simulink model "cmult_core"  (R2013a)
settings: Solver=ode45  StartTime=0.0  StopTime=10.0  RelTol=1e-3
libraries: xbsIndex_r4 x2035, casper_library_misc x116, casper_library_multipliers x36
(part 2 of 23)

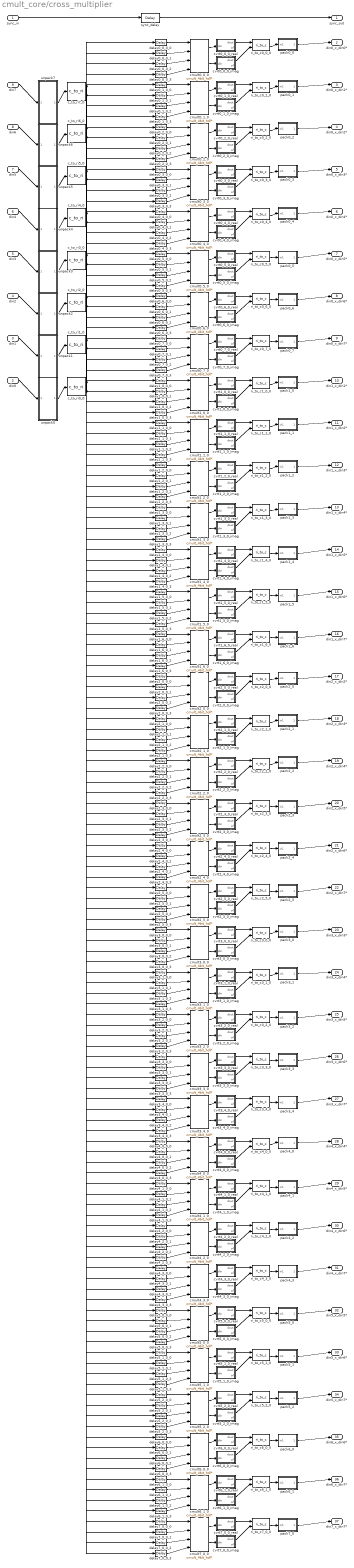
== system cmult_core/cross_multiplier ==
  sync_in : Inport
  din0 : Inport  Port=2
  din1 : Inport  Port=3
  din2 : Inport  Port=4
  din3 : Inport  Port=5
  din4 : Inport  Port=6
  din5 : Inport  Port=7
  din6 : Inport  Port=8
  din7 : Inport  Port=9
  c_to_ri0_0 : casper_library_misc/c_to_ri  n_bits=bit_width_in  bin_pt=binary_point_in
      settings: AttributesFormatString=8_7 r/i
  c_to_ri1_0 : casper_library_misc/c_to_ri  n_bits=bit_width_in  bin_pt=binary_point_in
      settings: AttributesFormatString=8_7 r/i
  c_to_ri2_0 : casper_library_misc/c_to_ri  n_bits=bit_width_in  bin_pt=binary_point_in
      settings: AttributesFormatString=8_7 r/i
  c_to_ri3_0 : casper_library_misc/c_to_ri  n_bits=bit_width_in  bin_pt=binary_point_in
      settings: AttributesFormatString=8_7 r/i
  c_to_ri4_0 : casper_library_misc/c_to_ri  n_bits=bit_width_in  bin_pt=binary_point_in
      settings: AttributesFormatString=8_7 r/i
  c_to_ri5_0 : casper_library_misc/c_to_ri  n_bits=bit_width_in  bin_pt=binary_point_in
      settings: AttributesFormatString=8_7 r/i
  c_to_ri6_0 : casper_library_misc/c_to_ri  n_bits=bit_width_in  bin_pt=binary_point_in
      settings: AttributesFormatString=8_7 r/i
  c_to_ri7_0 : casper_library_misc/c_to_ri  n_bits=bit_width_in  bin_pt=binary_point_in
      settings: AttributesFormatString=8_7 r/i
  cmult0_0_0 : casper_library_multipliers/cmult_4bit_hdl*  mult_latency=mult_latency  add_latency=add_latency
  cmult0_1_0 : casper_library_multipliers/cmult_4bit_hdl*  mult_latency=mult_latency  add_latency=add_latency
  cmult0_2_0 : casper_library_multipliers/cmult_4bit_hdl*  mult_latency=mult_latency  add_latency=add_latency
  cmult0_3_0 : casper_library_multipliers/cmult_4bit_hdl*  mult_latency=mult_latency  add_latency=add_latency
  cmult0_4_0 : casper_library_multipliers/cmult_4bit_hdl*  mult_latency=mult_latency  add_latency=add_latency
  cmult0_5_0 : casper_library_multipliers/cmult_4bit_hdl*  mult_latency=mult_latency  add_latency=add_latency
  cmult0_6_0 : casper_library_multipliers/cmult_4bit_hdl*  mult_latency=mult_latency  add_latency=add_latency
  cmult0_7_0 : casper_library_multipliers/cmult_4bit_hdl*  mult_latency=mult_latency  add_latency=add_latency
  cmult1_0_0 : casper_library_multipliers/cmult_4bit_hdl*  mult_latency=mult_latency  add_latency=add_latency
  cmult1_1_0 : casper_library_multipliers/cmult_4bit_hdl*  mult_latency=mult_latency  add_latency=add_latency
  cmult1_2_0 : casper_library_multipliers/cmult_4bit_hdl*  mult_latency=mult_latency  add_latency=add_latency
  cmult1_3_0 : casper_library_multipliers/cmult_4bit_hdl*  mult_latency=mult_latency  add_latency=add_latency
  cmult1_4_0 : casper_library_multipliers/cmult_4bit_hdl*  mult_latency=mult_latency  add_latency=add_latency
  cmult1_5_0 : casper_library_multipliers/cmult_4bit_hdl*  mult_latency=mult_latency  add_latency=add_latency
  cmult1_6_0 : casper_library_multipliers/cmult_4bit_hdl*  mult_latency=mult_latency  add_latency=add_latency
  cmult2_0_0 : casper_library_multipliers/cmult_4bit_hdl*  mult_latency=mult_latency  add_latency=add_latency
  cmult2_1_0 : casper_library_multipliers/cmult_4bit_hdl*  mult_latency=mult_latency  add_latency=add_latency
  cmult2_2_0 : casper_library_multipliers/cmult_4bit_hdl*  mult_latency=mult_latency  add_latency=add_latency
  cmult2_3_0 : casper_library_multipliers/cmult_4bit_hdl*  mult_latency=mult_latency  add_latency=add_latency
  cmult2_4_0 : casper_library_multipliers/cmult_4bit_hdl*  mult_latency=mult_latency  add_latency=add_latency
  cmult2_5_0 : casper_library_multipliers/cmult_4bit_hdl*  mult_latency=mult_latency  add_latency=add_latency
  cmult3_0_0 : casper_library_multipliers/cmult_4bit_hdl*  mult_latency=mult_latency  add_latency=add_latency
  cmult3_1_0 : casper_library_multipliers/cmult_4bit_hdl*  mult_latency=mult_latency  add_latency=add_latency
  cmult3_2_0 : casper_library_multipliers/cmult_4bit_hdl*  mult_latency=mult_latency  add_latency=add_latency
  cmult3_3_0 : casper_library_multipliers/cmult_4bit_hdl*  mult_latency=mult_latency  add_latency=add_latency
  cmult3_4_0 : casper_library_multipliers/cmult_4bit_hdl*  mult_latency=mult_latency  add_latency=add_latency
  cmult4_0_0 : casper_library_multipliers/cmult_4bit_hdl*  mult_latency=mult_latency  add_latency=add_latency
  cmult4_1_0 : casper_library_multipliers/cmult_4bit_hdl*  mult_latency=mult_latency  add_latency=add_latency
  cmult4_2_0 : casper_library_multipliers/cmult_4bit_hdl*  mult_latency=mult_latency  add_latency=add_latency
  cmult4_3_0 : casper_library_multipliers/cmult_4bit_hdl*  mult_latency=mult_latency  add_latency=add_latency
  cmult5_0_0 : casper_library_multipliers/cmult_4bit_hdl*  mult_latency=mult_latency  add_latency=add_latency
  cmult5_1_0 : casper_library_multipliers/cmult_4bit_hdl*  mult_latency=mult_latency  add_latency=add_latency
  cmult5_2_0 : casper_library_multipliers/cmult_4bit_hdl*  mult_latency=mult_latency  add_latency=add_latency
  cmult6_0_0 : casper_library_multipliers/cmult_4bit_hdl*  mult_latency=mult_latency  add_latency=add_latency
  cmult6_1_0 : casper_library_multipliers/cmult_4bit_hdl*  mult_latency=mult_latency  add_latency=add_latency
  cmult7_0_0 : casper_library_multipliers/cmult_4bit_hdl*  mult_latency=mult_latency  add_latency=add_latency
  cvrt0_0_0_imag : Subsystem  AncestorBlock=casper_library_misc/convert_of  mask(convert_of){bit_width_i=17, binary_point_i=14, bit_width_o=17, binary_point_o=14, latency=0, adder_imp=Fabric, overflow=Wrap, quantization=Truncate}
      mask prompts: bit_width_i "Bit Width In"; binary_point_i "Binary Point In"; bit_width_o "Bit Width Out"; binary_point_o "Binary Point Out"; adder_imp "Adder Implementation"; overflow "Overflow Behaviour"; quantization "Quantization Behaviour"
      mask help:
      | Converts from one 2's complement bit-width
      | and/or binary point position to another.
      | Includes underflow/overflow indicator.
      mask init:
      | convert_of_init(gcb, ...
      |     'bit_width_i', bit_width_i, ...
      |     'binary_point_i', binary_point_i, ...
      |     'bit_width_o', bit_width_o, ...
      |     'binary_point_o', binary_point_o, ...
      |     'latency', latency, ...
      |     'adder_imp', adder_imp, ...
      |     'overflow', overflow, ...
      |     'quantization', quantization);
      settings: AttributesFormatString=[17,14]->[17,14]
      mask TypeOptions adder_imp: Fabric | DSP48 | Behavioural | Xilinx Cast Block
      mask TypeOptions overflow: Wrap | Saturate | Error
      mask TypeOptions quantization: Truncate | Round  (unbiased: +/- Inf) | Round  (unbiased: even values)
  cvrt0_0_0_real : Subsystem  AncestorBlock=casper_library_misc/convert_of  mask(convert_of){bit_width_i=17, binary_point_i=14, bit_width_o=17, binary_point_o=14, latency=0, adder_imp=Fabric, overflow=Wrap, quantization=Truncate}
      mask prompts: bit_width_i "Bit Width In"; binary_point_i "Binary Point In"; bit_width_o "Bit Width Out"; binary_point_o "Binary Point Out"; adder_imp "Adder Implementation"; overflow "Overflow Behaviour"; quantization "Quantization Behaviour"
      mask help:
      | Converts from one 2's complement bit-width
      | and/or binary point position to another.
      | Includes underflow/overflow indicator.
      mask init: same as cmult_core/cross_multiplier/cvrt0_0_0_imag
      settings: AttributesFormatString=[17,14]->[17,14]
      mask TypeOptions adder_imp: Fabric | DSP48 | Behavioural | Xilinx Cast Block
      mask TypeOptions overflow: Wrap | Saturate | Error
      mask TypeOptions quantization: Truncate | Round  (unbiased: +/- Inf) | Round  (unbiased: even values)
  cvrt0_1_0_imag : Subsystem  AncestorBlock=casper_library_misc/convert_of  mask(convert_of){bit_width_i=17, binary_point_i=14, bit_width_o=17, binary_point_o=14, latency=0, adder_imp=Fabric, overflow=Wrap, quantization=Truncate}
      mask prompts: bit_width_i "Bit Width In"; binary_point_i "Binary Point In"; bit_width_o "Bit Width Out"; binary_point_o "Binary Point Out"; adder_imp "Adder Implementation"; overflow "Overflow Behaviour"; quantization "Quantization Behaviour"
      mask help:
      | Converts from one 2's complement bit-width
      | and/or binary point position to another.
      | Includes underflow/overflow indicator.
      mask init: same as cmult_core/cross_multiplier/cvrt0_0_0_imag
      settings: AttributesFormatString=[17,14]->[17,14]
      mask TypeOptions adder_imp: Fabric | DSP48 | Behavioural | Xilinx Cast Block
      mask TypeOptions overflow: Wrap | Saturate | Error
      mask TypeOptions quantization: Truncate | Round  (unbiased: +/- Inf) | Round  (unbiased: even values)
  cvrt0_1_0_real : Subsystem  AncestorBlock=casper_library_misc/convert_of  mask(convert_of){bit_width_i=17, binary_point_i=14, bit_width_o=17, binary_point_o=14, latency=0, adder_imp=Fabric, overflow=Wrap, quantization=Truncate}
      mask prompts: bit_width_i "Bit Width In"; binary_point_i "Binary Point In"; bit_width_o "Bit Width Out"; binary_point_o "Binary Point Out"; adder_imp "Adder Implementation"; overflow "Overflow Behaviour"; quantization "Quantization Behaviour"
      mask help:
      | Converts from one 2's complement bit-width
      | and/or binary point position to another.
      | Includes underflow/overflow indicator.
      mask init: same as cmult_core/cross_multiplier/cvrt0_0_0_imag
      settings: AttributesFormatString=[17,14]->[17,14]
      mask TypeOptions adder_imp: Fabric | DSP48 | Behavioural | Xilinx Cast Block
      mask TypeOptions overflow: Wrap | Saturate | Error
      mask TypeOptions quantization: Truncate | Round  (unbiased: +/- Inf) | Round  (unbiased: even values)
  cvrt0_2_0_imag : Subsystem  AncestorBlock=casper_library_misc/convert_of  mask(convert_of){bit_width_i=17, binary_point_i=14, bit_width_o=17, binary_point_o=14, latency=0, adder_imp=Fabric, overflow=Wrap, quantization=Truncate}
      mask prompts: bit_width_i "Bit Width In"; binary_point_i "Binary Point In"; bit_width_o "Bit Width Out"; binary_point_o "Binary Point Out"; adder_imp "Adder Implementation"; overflow "Overflow Behaviour"; quantization "Quantization Behaviour"
      mask help:
      | Converts from one 2's complement bit-width
      | and/or binary point position to another.
      | Includes underflow/overflow indicator.
      mask init: same as cmult_core/cross_multiplier/cvrt0_0_0_imag
      settings: AttributesFormatString=[17,14]->[17,14]
      mask TypeOptions adder_imp: Fabric | DSP48 | Behavioural | Xilinx Cast Block
      mask TypeOptions overflow: Wrap | Saturate | Error
      mask TypeOptions quantization: Truncate | Round  (unbiased: +/- Inf) | Round  (unbiased: even values)
  cvrt0_2_0_real : Subsystem  AncestorBlock=casper_library_misc/convert_of  mask(convert_of){bit_width_i=17, binary_point_i=14, bit_width_o=17, binary_point_o=14, latency=0, adder_imp=Fabric, overflow=Wrap, quantization=Truncate}
      mask prompts: bit_width_i "Bit Width In"; binary_point_i "Binary Point In"; bit_width_o "Bit Width Out"; binary_point_o "Binary Point Out"; adder_imp "Adder Implementation"; overflow "Overflow Behaviour"; quantization "Quantization Behaviour"
      mask help:
      | Converts from one 2's complement bit-width
      | and/or binary point position to another.
      | Includes underflow/overflow indicator.
      mask init: same as cmult_core/cross_multiplier/cvrt0_0_0_imag
      settings: AttributesFormatString=[17,14]->[17,14]
      mask TypeOptions adder_imp: Fabric | DSP48 | Behavioural | Xilinx Cast Block
      mask TypeOptions overflow: Wrap | Saturate | Error
      mask TypeOptions quantization: Truncate | Round  (unbiased: +/- Inf) | Round  (unbiased: even values)
  cvrt0_3_0_imag : Subsystem  AncestorBlock=casper_library_misc/convert_of  mask(convert_of){bit_width_i=17, binary_point_i=14, bit_width_o=17, binary_point_o=14, latency=0, adder_imp=Fabric, overflow=Wrap, quantization=Truncate}
      mask prompts: bit_width_i "Bit Width In"; binary_point_i "Binary Point In"; bit_width_o "Bit Width Out"; binary_point_o "Binary Point Out"; adder_imp "Adder Implementation"; overflow "Overflow Behaviour"; quantization "Quantization Behaviour"
      mask help:
      | Converts from one 2's complement bit-width
      | and/or binary point position to another.
      | Includes underflow/overflow indicator.
      mask init: same as cmult_core/cross_multiplier/cvrt0_0_0_imag
      settings: AttributesFormatString=[17,14]->[17,14]
      mask TypeOptions adder_imp: Fabric | DSP48 | Behavioural | Xilinx Cast Block
      mask TypeOptions overflow: Wrap | Saturate | Error
      mask TypeOptions quantization: Truncate | Round  (unbiased: +/- Inf) | Round  (unbiased: even values)
  cvrt0_3_0_real : Subsystem  AncestorBlock=casper_library_misc/convert_of  mask(convert_of){bit_width_i=17, binary_point_i=14, bit_width_o=17, binary_point_o=14, latency=0, adder_imp=Fabric, overflow=Wrap, quantization=Truncate}
      mask prompts: bit_width_i "Bit Width In"; binary_point_i "Binary Point In"; bit_width_o "Bit Width Out"; binary_point_o "Binary Point Out"; adder_imp "Adder Implementation"; overflow "Overflow Behaviour"; quantization "Quantization Behaviour"
      mask help:
      | Converts from one 2's complement bit-width
      | and/or binary point position to another.
      | Includes underflow/overflow indicator.
      mask init: same as cmult_core/cross_multiplier/cvrt0_0_0_imag
      settings: AttributesFormatString=[17,14]->[17,14]
      mask TypeOptions adder_imp: Fabric | DSP48 | Behavioural | Xilinx Cast Block
      mask TypeOptions overflow: Wrap | Saturate | Error
      mask TypeOptions quantization: Truncate | Round  (unbiased: +/- Inf) | Round  (unbiased: even values)
  cvrt0_4_0_imag : Subsystem  AncestorBlock=casper_library_misc/convert_of  mask(convert_of){bit_width_i=17, binary_point_i=14, bit_width_o=17, binary_point_o=14, latency=0, adder_imp=Fabric, overflow=Wrap, quantization=Truncate}
      mask prompts: bit_width_i "Bit Width In"; binary_point_i "Binary Point In"; bit_width_o "Bit Width Out"; binary_point_o "Binary Point Out"; adder_imp "Adder Implementation"; overflow "Overflow Behaviour"; quantization "Quantization Behaviour"
      mask help:
      | Converts from one 2's complement bit-width
      | and/or binary point position to another.
      | Includes underflow/overflow indicator.
      mask init: same as cmult_core/cross_multiplier/cvrt0_0_0_imag
      settings: AttributesFormatString=[17,14]->[17,14]
      mask TypeOptions adder_imp: Fabric | DSP48 | Behavioural | Xilinx Cast Block
      mask TypeOptions overflow: Wrap | Saturate | Error
      mask TypeOptions quantization: Truncate | Round  (unbiased: +/- Inf) | Round  (unbiased: even values)
  cvrt0_4_0_real : Subsystem  AncestorBlock=casper_library_misc/convert_of  mask(convert_of){bit_width_i=17, binary_point_i=14, bit_width_o=17, binary_point_o=14, latency=0, adder_imp=Fabric, overflow=Wrap, quantization=Truncate}
      mask prompts: bit_width_i "Bit Width In"; binary_point_i "Binary Point In"; bit_width_o "Bit Width Out"; binary_point_o "Binary Point Out"; adder_imp "Adder Implementation"; overflow "Overflow Behaviour"; quantization "Quantization Behaviour"
      mask help:
      | Converts from one 2's complement bit-width
      | and/or binary point position to another.
      | Includes underflow/overflow indicator.
      mask init: same as cmult_core/cross_multiplier/cvrt0_0_0_imag
      settings: AttributesFormatString=[17,14]->[17,14]
      mask TypeOptions adder_imp: Fabric | DSP48 | Behavioural | Xilinx Cast Block
      mask TypeOptions overflow: Wrap | Saturate | Error
      mask TypeOptions quantization: Truncate | Round  (unbiased: +/- Inf) | Round  (unbiased: even values)
  cvrt0_5_0_imag : Subsystem  AncestorBlock=casper_library_misc/convert_of  mask(convert_of){bit_width_i=17, binary_point_i=14, bit_width_o=17, binary_point_o=14, latency=0, adder_imp=Fabric, overflow=Wrap, quantization=Truncate}
      mask prompts: bit_width_i "Bit Width In"; binary_point_i "Binary Point In"; bit_width_o "Bit Width Out"; binary_point_o "Binary Point Out"; adder_imp "Adder Implementation"; overflow "Overflow Behaviour"; quantization "Quantization Behaviour"
      mask help:
      | Converts from one 2's complement bit-width
      | and/or binary point position to another.
      | Includes underflow/overflow indicator.
      mask init: same as cmult_core/cross_multiplier/cvrt0_0_0_imag
      settings: AttributesFormatString=[17,14]->[17,14]
      mask TypeOptions adder_imp: Fabric | DSP48 | Behavioural | Xilinx Cast Block
      mask TypeOptions overflow: Wrap | Saturate | Error
      mask TypeOptions quantization: Truncate | Round  (unbiased: +/- Inf) | Round  (unbiased: even values)
  cvrt0_5_0_real : Subsystem  AncestorBlock=casper_library_misc/convert_of  mask(convert_of){bit_width_i=17, binary_point_i=14, bit_width_o=17, binary_point_o=14, latency=0, adder_imp=Fabric, overflow=Wrap, quantization=Truncate}
      mask prompts: bit_width_i "Bit Width In"; binary_point_i "Binary Point In"; bit_width_o "Bit Width Out"; binary_point_o "Binary Point Out"; adder_imp "Adder Implementation"; overflow "Overflow Behaviour"; quantization "Quantization Behaviour"
      mask help:
      | Converts from one 2's complement bit-width
      | and/or binary point position to another.
      | Includes underflow/overflow indicator.
      mask init: same as cmult_core/cross_multiplier/cvrt0_0_0_imag
      settings: AttributesFormatString=[17,14]->[17,14]
      mask TypeOptions adder_imp: Fabric | DSP48 | Behavioural | Xilinx Cast Block
      mask TypeOptions overflow: Wrap | Saturate | Error
      mask TypeOptions quantization: Truncate | Round  (unbiased: +/- Inf) | Round  (unbiased: even values)
  cvrt0_6_0_imag : Subsystem  AncestorBlock=casper_library_misc/convert_of  mask(convert_of){bit_width_i=17, binary_point_i=14, bit_width_o=17, binary_point_o=14, latency=0, adder_imp=Fabric, overflow=Wrap, quantization=Truncate}
      mask prompts: bit_width_i "Bit Width In"; binary_point_i "Binary Point In"; bit_width_o "Bit Width Out"; binary_point_o "Binary Point Out"; adder_imp "Adder Implementation"; overflow "Overflow Behaviour"; quantization "Quantization Behaviour"
      mask help:
      | Converts from one 2's complement bit-width
      | and/or binary point position to another.
      | Includes underflow/overflow indicator.
      mask init: same as cmult_core/cross_multiplier/cvrt0_0_0_imag
      settings: AttributesFormatString=[17,14]->[17,14]
      mask TypeOptions adder_imp: Fabric | DSP48 | Behavioural | Xilinx Cast Block
      mask TypeOptions overflow: Wrap | Saturate | Error
      mask TypeOptions quantization: Truncate | Round  (unbiased: +/- Inf) | Round  (unbiased: even values)
  cvrt0_6_0_real : Subsystem  AncestorBlock=casper_library_misc/convert_of  mask(convert_of){bit_width_i=17, binary_point_i=14, bit_width_o=17, binary_point_o=14, latency=0, adder_imp=Fabric, overflow=Wrap, quantization=Truncate}
      mask prompts: bit_width_i "Bit Width In"; binary_point_i "Binary Point In"; bit_width_o "Bit Width Out"; binary_point_o "Binary Point Out"; adder_imp "Adder Implementation"; overflow "Overflow Behaviour"; quantization "Quantization Behaviour"
      mask help:
      | Converts from one 2's complement bit-width
      | and/or binary point position to another.
      | Includes underflow/overflow indicator.
      mask init: same as cmult_core/cross_multiplier/cvrt0_0_0_imag
      settings: AttributesFormatString=[17,14]->[17,14]
      mask TypeOptions adder_imp: Fabric | DSP48 | Behavioural | Xilinx Cast Block
      mask TypeOptions overflow: Wrap | Saturate | Error
      mask TypeOptions quantization: Truncate | Round  (unbiased: +/- Inf) | Round  (unbiased: even values)
  cvrt0_7_0_imag : Subsystem  AncestorBlock=casper_library_misc/convert_of  mask(convert_of){bit_width_i=17, binary_point_i=14, bit_width_o=17, binary_point_o=14, latency=0, adder_imp=Fabric, overflow=Wrap, quantization=Truncate}
      mask prompts: bit_width_i "Bit Width In"; binary_point_i "Binary Point In"; bit_width_o "Bit Width Out"; binary_point_o "Binary Point Out"; adder_imp "Adder Implementation"; overflow "Overflow Behaviour"; quantization "Quantization Behaviour"
      mask help:
      | Converts from one 2's complement bit-width
      | and/or binary point position to another.
      | Includes underflow/overflow indicator.
      mask init: same as cmult_core/cross_multiplier/cvrt0_0_0_imag
      settings: AttributesFormatString=[17,14]->[17,14]
      mask TypeOptions adder_imp: Fabric | DSP48 | Behavioural | Xilinx Cast Block
      mask TypeOptions overflow: Wrap | Saturate | Error
      mask TypeOptions quantization: Truncate | Round  (unbiased: +/- Inf) | Round  (unbiased: even values)
  cvrt0_7_0_real : Subsystem  AncestorBlock=casper_library_misc/convert_of  mask(convert_of){bit_width_i=17, binary_point_i=14, bit_width_o=17, binary_point_o=14, latency=0, adder_imp=Fabric, overflow=Wrap, quantization=Truncate}
      mask prompts: bit_width_i "Bit Width In"; binary_point_i "Binary Point In"; bit_width_o "Bit Width Out"; binary_point_o "Binary Point Out"; adder_imp "Adder Implementation"; overflow "Overflow Behaviour"; quantization "Quantization Behaviour"
      mask help:
      | Converts from one 2's complement bit-width
      | and/or binary point position to another.
      | Includes underflow/overflow indicator.
      mask init: same as cmult_core/cross_multiplier/cvrt0_0_0_imag
      settings: AttributesFormatString=[17,14]->[17,14]
      mask TypeOptions adder_imp: Fabric | DSP48 | Behavioural | Xilinx Cast Block
      mask TypeOptions overflow: Wrap | Saturate | Error
      mask TypeOptions quantization: Truncate | Round  (unbiased: +/- Inf) | Round  (unbiased: even values)
  cvrt1_0_0_imag : Subsystem  AncestorBlock=casper_library_misc/convert_of  mask(convert_of){bit_width_i=17, binary_point_i=14, bit_width_o=17, binary_point_o=14, latency=0, adder_imp=Fabric, overflow=Wrap, quantization=Truncate}
      mask prompts: bit_width_i "Bit Width In"; binary_point_i "Binary Point In"; bit_width_o "Bit Width Out"; binary_point_o "Binary Point Out"; adder_imp "Adder Implementation"; overflow "Overflow Behaviour"; quantization "Quantization Behaviour"
      mask help:
      | Converts from one 2's complement bit-width
      | and/or binary point position to another.
      | Includes underflow/overflow indicator.
      mask init: same as cmult_core/cross_multiplier/cvrt0_0_0_imag
      settings: AttributesFormatString=[17,14]->[17,14]
      mask TypeOptions adder_imp: Fabric | DSP48 | Behavioural | Xilinx Cast Block
      mask TypeOptions overflow: Wrap | Saturate | Error
      mask TypeOptions quantization: Truncate | Round  (unbiased: +/- Inf) | Round  (unbiased: even values)
  cvrt1_0_0_real : Subsystem  AncestorBlock=casper_library_misc/convert_of  mask(convert_of){bit_width_i=17, binary_point_i=14, bit_width_o=17, binary_point_o=14, latency=0, adder_imp=Fabric, overflow=Wrap, quantization=Truncate}
      mask prompts: bit_width_i "Bit Width In"; binary_point_i "Binary Point In"; bit_width_o "Bit Width Out"; binary_point_o "Binary Point Out"; adder_imp "Adder Implementation"; overflow "Overflow Behaviour"; quantization "Quantization Behaviour"
      mask help:
      | Converts from one 2's complement bit-width
      | and/or binary point position to another.
      | Includes underflow/overflow indicator.
      mask init: same as cmult_core/cross_multiplier/cvrt0_0_0_imag
      settings: AttributesFormatString=[17,14]->[17,14]
      mask TypeOptions adder_imp: Fabric | DSP48 | Behavioural | Xilinx Cast Block
      mask TypeOptions overflow: Wrap | Saturate | Error
      mask TypeOptions quantization: Truncate | Round  (unbiased: +/- Inf) | Round  (unbiased: even values)
  cvrt1_1_0_imag : Subsystem  AncestorBlock=casper_library_misc/convert_of  mask(convert_of){bit_width_i=17, binary_point_i=14, bit_width_o=17, binary_point_o=14, latency=0, adder_imp=Fabric, overflow=Wrap, quantization=Truncate}
      mask prompts: bit_width_i "Bit Width In"; binary_point_i "Binary Point In"; bit_width_o "Bit Width Out"; binary_point_o "Binary Point Out"; adder_imp "Adder Implementation"; overflow "Overflow Behaviour"; quantization "Quantization Behaviour"
      mask help:
      | Converts from one 2's complement bit-width
      | and/or binary point position to another.
      | Includes underflow/overflow indicator.
      mask init: same as cmult_core/cross_multiplier/cvrt0_0_0_imag
      settings: AttributesFormatString=[17,14]->[17,14]
      mask TypeOptions adder_imp: Fabric | DSP48 | Behavioural | Xilinx Cast Block
      mask TypeOptions overflow: Wrap | Saturate | Error
      mask TypeOptions quantization: Truncate | Round  (unbiased: +/- Inf) | Round  (unbiased: even values)
  cvrt1_1_0_real : Subsystem  AncestorBlock=casper_library_misc/convert_of  mask(convert_of){bit_width_i=17, binary_point_i=14, bit_width_o=17, binary_point_o=14, latency=0, adder_imp=Fabric, overflow=Wrap, quantization=Truncate}
      mask prompts: bit_width_i "Bit Width In"; binary_point_i "Binary Point In"; bit_width_o "Bit Width Out"; binary_point_o "Binary Point Out"; adder_imp "Adder Implementation"; overflow "Overflow Behaviour"; quantization "Quantization Behaviour"
      mask help:
      | Converts from one 2's complement bit-width
      | and/or binary point position to another.
      | Includes underflow/overflow indicator.
      mask init: same as cmult_core/cross_multiplier/cvrt0_0_0_imag
      settings: AttributesFormatString=[17,14]->[17,14]
      mask TypeOptions adder_imp: Fabric | DSP48 | Behavioural | Xilinx Cast Block
      mask TypeOptions overflow: Wrap | Saturate | Error
      mask TypeOptions quantization: Truncate | Round  (unbiased: +/- Inf) | Round  (unbiased: even values)
  cvrt1_2_0_imag : Subsystem  AncestorBlock=casper_library_misc/convert_of  mask(convert_of){bit_width_i=17, binary_point_i=14, bit_width_o=17, binary_point_o=14, latency=0, adder_imp=Fabric, overflow=Wrap, quantization=Truncate}
      mask prompts: bit_width_i "Bit Width In"; binary_point_i "Binary Point In"; bit_width_o "Bit Width Out"; binary_point_o "Binary Point Out"; adder_imp "Adder Implementation"; overflow "Overflow Behaviour"; quantization "Quantization Behaviour"
      mask help:
      | Converts from one 2's complement bit-width
      | and/or binary point position to another.
      | Includes underflow/overflow indicator.
      mask init: same as cmult_core/cross_multiplier/cvrt0_0_0_imag
      settings: AttributesFormatString=[17,14]->[17,14]
      mask TypeOptions adder_imp: Fabric | DSP48 | Behavioural | Xilinx Cast Block
      mask TypeOptions overflow: Wrap | Saturate | Error
      mask TypeOptions quantization: Truncate | Round  (unbiased: +/- Inf) | Round  (unbiased: even values)
  cvrt1_2_0_real : Subsystem  AncestorBlock=casper_library_misc/convert_of  mask(convert_of){bit_width_i=17, binary_point_i=14, bit_width_o=17, binary_point_o=14, latency=0, adder_imp=Fabric, overflow=Wrap, quantization=Truncate}
      mask prompts: bit_width_i "Bit Width In"; binary_point_i "Binary Point In"; bit_width_o "Bit Width Out"; binary_point_o "Binary Point Out"; adder_imp "Adder Implementation"; overflow "Overflow Behaviour"; quantization "Quantization Behaviour"
      mask help:
      | Converts from one 2's complement bit-width
      | and/or binary point position to another.
      | Includes underflow/overflow indicator.
      mask init: same as cmult_core/cross_multiplier/cvrt0_0_0_imag
      settings: AttributesFormatString=[17,14]->[17,14]
      mask TypeOptions adder_imp: Fabric | DSP48 | Behavioural | Xilinx Cast Block
      mask TypeOptions overflow: Wrap | Saturate | Error
      mask TypeOptions quantization: Truncate | Round  (unbiased: +/- Inf) | Round  (unbiased: even values)
  cvrt1_3_0_imag : Subsystem  AncestorBlock=casper_library_misc/convert_of  mask(convert_of){bit_width_i=17, binary_point_i=14, bit_width_o=17, binary_point_o=14, latency=0, adder_imp=Fabric, overflow=Wrap, quantization=Truncate}
      mask prompts: bit_width_i "Bit Width In"; binary_point_i "Binary Point In"; bit_width_o "Bit Width Out"; binary_point_o "Binary Point Out"; adder_imp "Adder Implementation"; overflow "Overflow Behaviour"; quantization "Quantization Behaviour"
      mask help:
      | Converts from one 2's complement bit-width
      | and/or binary point position to another.
      | Includes underflow/overflow indicator.
      mask init: same as cmult_core/cross_multiplier/cvrt0_0_0_imag
      settings: AttributesFormatString=[17,14]->[17,14]
      mask TypeOptions adder_imp: Fabric | DSP48 | Behavioural | Xilinx Cast Block
      mask TypeOptions overflow: Wrap | Saturate | Error
      mask TypeOptions quantization: Truncate | Round  (unbiased: +/- Inf) | Round  (unbiased: even values)
  cvrt1_3_0_real : Subsystem  AncestorBlock=casper_library_misc/convert_of  mask(convert_of){bit_width_i=17, binary_point_i=14, bit_width_o=17, binary_point_o=14, latency=0, adder_imp=Fabric, overflow=Wrap, quantization=Truncate}
      mask prompts: bit_width_i "Bit Width In"; binary_point_i "Binary Point In"; bit_width_o "Bit Width Out"; binary_point_o "Binary Point Out"; adder_imp "Adder Implementation"; overflow "Overflow Behaviour"; quantization "Quantization Behaviour"
      mask help:
      | Converts from one 2's complement bit-width
      | and/or binary point position to another.
      | Includes underflow/overflow indicator.
      mask init: same as cmult_core/cross_multiplier/cvrt0_0_0_imag
      settings: AttributesFormatString=[17,14]->[17,14]
      mask TypeOptions adder_imp: Fabric | DSP48 | Behavioural | Xilinx Cast Block
      mask TypeOptions overflow: Wrap | Saturate | Error
      mask TypeOptions quantization: Truncate | Round  (unbiased: +/- Inf) | Round  (unbiased: even values)
  cvrt1_4_0_imag : Subsystem  AncestorBlock=casper_library_misc/convert_of  mask(convert_of){bit_width_i=17, binary_point_i=14, bit_width_o=17, binary_point_o=14, latency=0, adder_imp=Fabric, overflow=Wrap, quantization=Truncate}
      mask prompts: bit_width_i "Bit Width In"; binary_point_i "Binary Point In"; bit_width_o "Bit Width Out"; binary_point_o "Binary Point Out"; adder_imp "Adder Implementation"; overflow "Overflow Behaviour"; quantization "Quantization Behaviour"
      mask help:
      | Converts from one 2's complement bit-width
      | and/or binary point position to another.
      | Includes underflow/overflow indicator.
      mask init: same as cmult_core/cross_multiplier/cvrt0_0_0_imag
      settings: AttributesFormatString=[17,14]->[17,14]
      mask TypeOptions adder_imp: Fabric | DSP48 | Behavioural | Xilinx Cast Block
      mask TypeOptions overflow: Wrap | Saturate | Error
      mask TypeOptions quantization: Truncate | Round  (unbiased: +/- Inf) | Round  (unbiased: even values)
  cvrt1_4_0_real : Subsystem  AncestorBlock=casper_library_misc/convert_of  mask(convert_of){bit_width_i=17, binary_point_i=14, bit_width_o=17, binary_point_o=14, latency=0, adder_imp=Fabric, overflow=Wrap, quantization=Truncate}
      mask prompts: bit_width_i "Bit Width In"; binary_point_i "Binary Point In"; bit_width_o "Bit Width Out"; binary_point_o "Binary Point Out"; adder_imp "Adder Implementation"; overflow "Overflow Behaviour"; quantization "Quantization Behaviour"
      mask help:
      | Converts from one 2's complement bit-width
      | and/or binary point position to another.
      | Includes underflow/overflow indicator.
      mask init: same as cmult_core/cross_multiplier/cvrt0_0_0_imag
      settings: AttributesFormatString=[17,14]->[17,14]
      mask TypeOptions adder_imp: Fabric | DSP48 | Behavioural | Xilinx Cast Block
      mask TypeOptions overflow: Wrap | Saturate | Error
      mask TypeOptions quantization: Truncate | Round  (unbiased: +/- Inf) | Round  (unbiased: even values)
  cvrt1_5_0_imag : Subsystem  AncestorBlock=casper_library_misc/convert_of  mask(convert_of){bit_width_i=17, binary_point_i=14, bit_width_o=17, binary_point_o=14, latency=0, adder_imp=Fabric, overflow=Wrap, quantization=Truncate}
      mask prompts: bit_width_i "Bit Width In"; binary_point_i "Binary Point In"; bit_width_o "Bit Width Out"; binary_point_o "Binary Point Out"; adder_imp "Adder Implementation"; overflow "Overflow Behaviour"; quantization "Quantization Behaviour"
      mask help:
      | Converts from one 2's complement bit-width
      | and/or binary point position to another.
      | Includes underflow/overflow indicator.
      mask init: same as cmult_core/cross_multiplier/cvrt0_0_0_imag
      settings: AttributesFormatString=[17,14]->[17,14]
      mask TypeOptions adder_imp: Fabric | DSP48 | Behavioural | Xilinx Cast Block
      mask TypeOptions overflow: Wrap | Saturate | Error
      mask TypeOptions quantization: Truncate | Round  (unbiased: +/- Inf) | Round  (unbiased: even values)
  cvrt1_5_0_real : Subsystem  AncestorBlock=casper_library_misc/convert_of  mask(convert_of){bit_width_i=17, binary_point_i=14, bit_width_o=17, binary_point_o=14, latency=0, adder_imp=Fabric, overflow=Wrap, quantization=Truncate}
      mask prompts: bit_width_i "Bit Width In"; binary_point_i "Binary Point In"; bit_width_o "Bit Width Out"; binary_point_o "Binary Point Out"; adder_imp "Adder Implementation"; overflow "Overflow Behaviour"; quantization "Quantization Behaviour"
      mask help:
      | Converts from one 2's complement bit-width
      | and/or binary point position to another.
      | Includes underflow/overflow indicator.
      mask init: same as cmult_core/cross_multiplier/cvrt0_0_0_imag
      settings: AttributesFormatString=[17,14]->[17,14]
      mask TypeOptions adder_imp: Fabric | DSP48 | Behavioural | Xilinx Cast Block
      mask TypeOptions overflow: Wrap | Saturate | Error
      mask TypeOptions quantization: Truncate | Round  (unbiased: +/- Inf) | Round  (unbiased: even values)
  cvrt1_6_0_imag : Subsystem  AncestorBlock=casper_library_misc/convert_of  mask(convert_of){bit_width_i=17, binary_point_i=14, bit_width_o=17, binary_point_o=14, latency=0, adder_imp=Fabric, overflow=Wrap, quantization=Truncate}
      mask prompts: bit_width_i "Bit Width In"; binary_point_i "Binary Point In"; bit_width_o "Bit Width Out"; binary_point_o "Binary Point Out"; adder_imp "Adder Implementation"; overflow "Overflow Behaviour"; quantization "Quantization Behaviour"
      mask help:
      | Converts from one 2's complement bit-width
      | and/or binary point position to another.
      | Includes underflow/overflow indicator.
      mask init: same as cmult_core/cross_multiplier/cvrt0_0_0_imag
      settings: AttributesFormatString=[17,14]->[17,14]
      mask TypeOptions adder_imp: Fabric | DSP48 | Behavioural | Xilinx Cast Block
      mask TypeOptions overflow: Wrap | Saturate | Error
      mask TypeOptions quantization: Truncate | Round  (unbiased: +/- Inf) | Round  (unbiased: even values)
  cvrt1_6_0_real : Subsystem  AncestorBlock=casper_library_misc/convert_of  mask(convert_of){bit_width_i=17, binary_point_i=14, bit_width_o=17, binary_point_o=14, latency=0, adder_imp=Fabric, overflow=Wrap, quantization=Truncate}
      mask prompts: bit_width_i "Bit Width In"; binary_point_i "Binary Point In"; bit_width_o "Bit Width Out"; binary_point_o "Binary Point Out"; adder_imp "Adder Implementation"; overflow "Overflow Behaviour"; quantization "Quantization Behaviour"
      mask help:
      | Converts from one 2's complement bit-width
      | and/or binary point position to another.
      | Includes underflow/overflow indicator.
      mask init: same as cmult_core/cross_multiplier/cvrt0_0_0_imag
      settings: AttributesFormatString=[17,14]->[17,14]
      mask TypeOptions adder_imp: Fabric | DSP48 | Behavioural | Xilinx Cast Block
      mask TypeOptions overflow: Wrap | Saturate | Error
      mask TypeOptions quantization: Truncate | Round  (unbiased: +/- Inf) | Round  (unbiased: even values)
  cvrt2_0_0_imag : Subsystem  AncestorBlock=casper_library_misc/convert_of  mask(convert_of){bit_width_i=17, binary_point_i=14, bit_width_o=17, binary_point_o=14, latency=0, adder_imp=Fabric, overflow=Wrap, quantization=Truncate}
      mask prompts: bit_width_i "Bit Width In"; binary_point_i "Binary Point In"; bit_width_o "Bit Width Out"; binary_point_o "Binary Point Out"; adder_imp "Adder Implementation"; overflow "Overflow Behaviour"; quantization "Quantization Behaviour"
      mask help:
      | Converts from one 2's complement bit-width
      | and/or binary point position to another.
      | Includes underflow/overflow indicator.
      mask init: same as cmult_core/cross_multiplier/cvrt0_0_0_imag
      settings: AttributesFormatString=[17,14]->[17,14]
      mask TypeOptions adder_imp: Fabric | DSP48 | Behavioural | Xilinx Cast Block
      mask TypeOptions overflow: Wrap | Saturate | Error
      mask TypeOptions quantization: Truncate | Round  (unbiased: +/- Inf) | Round  (unbiased: even values)
  cvrt2_0_0_real : Subsystem  AncestorBlock=casper_library_misc/convert_of  mask(convert_of){bit_width_i=17, binary_point_i=14, bit_width_o=17, binary_point_o=14, latency=0, adder_imp=Fabric, overflow=Wrap, quantization=Truncate}
      mask prompts: bit_width_i "Bit Width In"; binary_point_i "Binary Point In"; bit_width_o "Bit Width Out"; binary_point_o "Binary Point Out"; adder_imp "Adder Implementation"; overflow "Overflow Behaviour"; quantization "Quantization Behaviour"
      mask help:
      | Converts from one 2's complement bit-width
      | and/or binary point position to another.
      | Includes underflow/overflow indicator.
      mask init: same as cmult_core/cross_multiplier/cvrt0_0_0_imag
      settings: AttributesFormatString=[17,14]->[17,14]
      mask TypeOptions adder_imp: Fabric | DSP48 | Behavioural | Xilinx Cast Block
      mask TypeOptions overflow: Wrap | Saturate | Error
      mask TypeOptions quantization: Truncate | Round  (unbiased: +/- Inf) | Round  (unbiased: even values)
  cvrt2_1_0_imag : Subsystem  AncestorBlock=casper_library_misc/convert_of  mask(convert_of){bit_width_i=17, binary_point_i=14, bit_width_o=17, binary_point_o=14, latency=0, adder_imp=Fabric, overflow=Wrap, quantization=Truncate}
      mask prompts: bit_width_i "Bit Width In"; binary_point_i "Binary Point In"; bit_width_o "Bit Width Out"; binary_point_o "Binary Point Out"; adder_imp "Adder Implementation"; overflow "Overflow Behaviour"; quantization "Quantization Behaviour"
      mask help:
      | Converts from one 2's complement bit-width
      | and/or binary point position to another.
      | Includes underflow/overflow indicator.
      mask init: same as cmult_core/cross_multiplier/cvrt0_0_0_imag
      settings: AttributesFormatString=[17,14]->[17,14]
      mask TypeOptions adder_imp: Fabric | DSP48 | Behavioural | Xilinx Cast Block
      mask TypeOptions overflow: Wrap | Saturate | Error
      mask TypeOptions quantization: Truncate | Round  (unbiased: +/- Inf) | Round  (unbiased: even values)
  cvrt2_1_0_real : Subsystem  AncestorBlock=casper_library_misc/convert_of  mask(convert_of){bit_width_i=17, binary_point_i=14, bit_width_o=17, binary_point_o=14, latency=0, adder_imp=Fabric, overflow=Wrap, quantization=Truncate}
      mask prompts: bit_width_i "Bit Width In"; binary_point_i "Binary Point In"; bit_width_o "Bit Width Out"; binary_point_o "Binary Point Out"; adder_imp "Adder Implementation"; overflow "Overflow Behaviour"; quantization "Quantization Behaviour"
      mask help:
      | Converts from one 2's complement bit-width
      | and/or binary point position to another.
      | Includes underflow/overflow indicator.
      mask init: same as cmult_core/cross_multiplier/cvrt0_0_0_imag
      settings: AttributesFormatString=[17,14]->[17,14]
      mask TypeOptions adder_imp: Fabric | DSP48 | Behavioural | Xilinx Cast Block
      mask TypeOptions overflow: Wrap | Saturate | Error
      mask TypeOptions quantization: Truncate | Round  (unbiased: +/- Inf) | Round  (unbiased: even values)
  cvrt2_2_0_imag : Subsystem  AncestorBlock=casper_library_misc/convert_of  mask(convert_of){bit_width_i=17, binary_point_i=14, bit_width_o=17, binary_point_o=14, latency=0, adder_imp=Fabric, overflow=Wrap, quantization=Truncate}
      mask prompts: bit_width_i "Bit Width In"; binary_point_i "Binary Point In"; bit_width_o "Bit Width Out"; binary_point_o "Binary Point Out"; adder_imp "Adder Implementation"; overflow "Overflow Behaviour"; quantization "Quantization Behaviour"
      mask help:
      | Converts from one 2's complement bit-width
      | and/or binary point position to another.
      | Includes underflow/overflow indicator.
      mask init: same as cmult_core/cross_multiplier/cvrt0_0_0_imag
      settings: AttributesFormatString=[17,14]->[17,14]
      mask TypeOptions adder_imp: Fabric | DSP48 | Behavioural | Xilinx Cast Block
      mask TypeOptions overflow: Wrap | Saturate | Error
      mask TypeOptions quantization: Truncate | Round  (unbiased: +/- Inf) | Round  (unbiased: even values)
  cvrt2_2_0_real : Subsystem  AncestorBlock=casper_library_misc/convert_of  mask(convert_of){bit_width_i=17, binary_point_i=14, bit_width_o=17, binary_point_o=14, latency=0, adder_imp=Fabric, overflow=Wrap, quantization=Truncate}
      mask prompts: bit_width_i "Bit Width In"; binary_point_i "Binary Point In"; bit_width_o "Bit Width Out"; binary_point_o "Binary Point Out"; adder_imp "Adder Implementation"; overflow "Overflow Behaviour"; quantization "Quantization Behaviour"
      mask help:
      | Converts from one 2's complement bit-width
      | and/or binary point position to another.
      | Includes underflow/overflow indicator.
      mask init: same as cmult_core/cross_multiplier/cvrt0_0_0_imag
      settings: AttributesFormatString=[17,14]->[17,14]
      mask TypeOptions adder_imp: Fabric | DSP48 | Behavioural | Xilinx Cast Block
      mask TypeOptions overflow: Wrap | Saturate | Error
      mask TypeOptions quantization: Truncate | Round  (unbiased: +/- Inf) | Round  (unbiased: even values)
  cvrt2_3_0_imag : Subsystem  AncestorBlock=casper_library_misc/convert_of  mask(convert_of){bit_width_i=17, binary_point_i=14, bit_width_o=17, binary_point_o=14, latency=0, adder_imp=Fabric, overflow=Wrap, quantization=Truncate}
      mask prompts: bit_width_i "Bit Width In"; binary_point_i "Binary Point In"; bit_width_o "Bit Width Out"; binary_point_o "Binary Point Out"; adder_imp "Adder Implementation"; overflow "Overflow Behaviour"; quantization "Quantization Behaviour"
      mask help:
      | Converts from one 2's complement bit-width
      | and/or binary point position to another.
      | Includes underflow/overflow indicator.
      mask init: same as cmult_core/cross_multiplier/cvrt0_0_0_imag
      settings: AttributesFormatString=[17,14]->[17,14]
      mask TypeOptions adder_imp: Fabric | DSP48 | Behavioural | Xilinx Cast Block
      mask TypeOptions overflow: Wrap | Saturate | Error
      mask TypeOptions quantization: Truncate | Round  (unbiased: +/- Inf) | Round  (unbiased: even values)
  cvrt2_3_0_real : Subsystem  AncestorBlock=casper_library_misc/convert_of  mask(convert_of){bit_width_i=17, binary_point_i=14, bit_width_o=17, binary_point_o=14, latency=0, adder_imp=Fabric, overflow=Wrap, quantization=Truncate}
      mask prompts: bit_width_i "Bit Width In"; binary_point_i "Binary Point In"; bit_width_o "Bit Width Out"; binary_point_o "Binary Point Out"; adder_imp "Adder Implementation"; overflow "Overflow Behaviour"; quantization "Quantization Behaviour"
      mask help:
      | Converts from one 2's complement bit-width
      | and/or binary point position to another.
      | Includes underflow/overflow indicator.
      mask init: same as cmult_core/cross_multiplier/cvrt0_0_0_imag
      settings: AttributesFormatString=[17,14]->[17,14]
      mask TypeOptions adder_imp: Fabric | DSP48 | Behavioural | Xilinx Cast Block
      mask TypeOptions overflow: Wrap | Saturate | Error
      mask TypeOptions quantization: Truncate | Round  (unbiased: +/- Inf) | Round  (unbiased: even values)
  cvrt2_4_0_imag : Subsystem  AncestorBlock=casper_library_misc/convert_of  mask(convert_of){bit_width_i=17, binary_point_i=14, bit_width_o=17, binary_point_o=14, latency=0, adder_imp=Fabric, overflow=Wrap, quantization=Truncate}
      mask prompts: bit_width_i "Bit Width In"; binary_point_i "Binary Point In"; bit_width_o "Bit Width Out"; binary_point_o "Binary Point Out"; adder_imp "Adder Implementation"; overflow "Overflow Behaviour"; quantization "Quantization Behaviour"
      mask help:
      | Converts from one 2's complement bit-width
      | and/or binary point position to another.
      | Includes underflow/overflow indicator.
      mask init: same as cmult_core/cross_multiplier/cvrt0_0_0_imag
      settings: AttributesFormatString=[17,14]->[17,14]
      mask TypeOptions adder_imp: Fabric | DSP48 | Behavioural | Xilinx Cast Block
      mask TypeOptions overflow: Wrap | Saturate | Error
      mask TypeOptions quantization: Truncate | Round  (unbiased: +/- Inf) | Round  (unbiased: even values)
  cvrt2_4_0_real : Subsystem  AncestorBlock=casper_library_misc/convert_of  mask(convert_of){bit_width_i=17, binary_point_i=14, bit_width_o=17, binary_point_o=14, latency=0, adder_imp=Fabric, overflow=Wrap, quantization=Truncate}
      mask prompts: bit_width_i "Bit Width In"; binary_point_i "Binary Point In"; bit_width_o "Bit Width Out"; binary_point_o "Binary Point Out"; adder_imp "Adder Implementation"; overflow "Overflow Behaviour"; quantization "Quantization Behaviour"
      mask help:
      | Converts from one 2's complement bit-width
      | and/or binary point position to another.
      | Includes underflow/overflow indicator.
      mask init: same as cmult_core/cross_multiplier/cvrt0_0_0_imag
      settings: AttributesFormatString=[17,14]->[17,14]
      mask TypeOptions adder_imp: Fabric | DSP48 | Behavioural | Xilinx Cast Block
      mask TypeOptions overflow: Wrap | Saturate | Error
      mask TypeOptions quantization: Truncate | Round  (unbiased: +/- Inf) | Round  (unbiased: even values)
  cvrt2_5_0_imag : Subsystem  AncestorBlock=casper_library_misc/convert_of  mask(convert_of){bit_width_i=17, binary_point_i=14, bit_width_o=17, binary_point_o=14, latency=0, adder_imp=Fabric, overflow=Wrap, quantization=Truncate}
      mask prompts: bit_width_i "Bit Width In"; binary_point_i "Binary Point In"; bit_width_o "Bit Width Out"; binary_point_o "Binary Point Out"; adder_imp "Adder Implementation"; overflow "Overflow Behaviour"; quantization "Quantization Behaviour"
      mask help:
      | Converts from one 2's complement bit-width
      | and/or binary point position to another.
      | Includes underflow/overflow indicator.
      mask init: same as cmult_core/cross_multiplier/cvrt0_0_0_imag
      settings: AttributesFormatString=[17,14]->[17,14]
      mask TypeOptions adder_imp: Fabric | DSP48 | Behavioural | Xilinx Cast Block
      mask TypeOptions overflow: Wrap | Saturate | Error
      mask TypeOptions quantization: Truncate | Round  (unbiased: +/- Inf) | Round  (unbiased: even values)
  cvrt2_5_0_real : Subsystem  AncestorBlock=casper_library_misc/convert_of  mask(convert_of){bit_width_i=17, binary_point_i=14, bit_width_o=17, binary_point_o=14, latency=0, adder_imp=Fabric, overflow=Wrap, quantization=Truncate}
      mask prompts: bit_width_i "Bit Width In"; binary_point_i "Binary Point In"; bit_width_o "Bit Width Out"; binary_point_o "Binary Point Out"; adder_imp "Adder Implementation"; overflow "Overflow Behaviour"; quantization "Quantization Behaviour"
      mask help:
      | Converts from one 2's complement bit-width
      | and/or binary point position to another.
      | Includes underflow/overflow indicator.
      mask init: same as cmult_core/cross_multiplier/cvrt0_0_0_imag
      settings: AttributesFormatString=[17,14]->[17,14]
      mask TypeOptions adder_imp: Fabric | DSP48 | Behavioural | Xilinx Cast Block
      mask TypeOptions overflow: Wrap | Saturate | Error
      mask TypeOptions quantization: Truncate | Round  (unbiased: +/- Inf) | Round  (unbiased: even values)
  cvrt3_0_0_imag : Subsystem  AncestorBlock=casper_library_misc/convert_of  mask(convert_of){bit_width_i=17, binary_point_i=14, bit_width_o=17, binary_point_o=14, latency=0, adder_imp=Fabric, overflow=Wrap, quantization=Truncate}
      mask prompts: bit_width_i "Bit Width In"; binary_point_i "Binary Point In"; bit_width_o "Bit Width Out"; binary_point_o "Binary Point Out"; adder_imp "Adder Implementation"; overflow "Overflow Behaviour"; quantization "Quantization Behaviour"
      mask help:
      | Converts from one 2's complement bit-width
      | and/or binary point position to another.
      | Includes underflow/overflow indicator.
      mask init: same as cmult_core/cross_multiplier/cvrt0_0_0_imag
      settings: AttributesFormatString=[17,14]->[17,14]
      mask TypeOptions adder_imp: Fabric | DSP48 | Behavioural | Xilinx Cast Block
      mask TypeOptions overflow: Wrap | Saturate | Error
      mask TypeOptions quantization: Truncate | Round  (unbiased: +/- Inf) | Round  (unbiased: even values)
  cvrt3_0_0_real : Subsystem  AncestorBlock=casper_library_misc/convert_of  mask(convert_of){bit_width_i=17, binary_point_i=14, bit_width_o=17, binary_point_o=14, latency=0, adder_imp=Fabric, overflow=Wrap, quantization=Truncate}
      mask prompts: bit_width_i "Bit Width In"; binary_point_i "Binary Point In"; bit_width_o "Bit Width Out"; binary_point_o "Binary Point Out"; adder_imp "Adder Implementation"; overflow "Overflow Behaviour"; quantization "Quantization Behaviour"
      mask help:
      | Converts from one 2's complement bit-width
      | and/or binary point position to another.
      | Includes underflow/overflow indicator.
      mask init: same as cmult_core/cross_multiplier/cvrt0_0_0_imag
      settings: AttributesFormatString=[17,14]->[17,14]
      mask TypeOptions adder_imp: Fabric | DSP48 | Behavioural | Xilinx Cast Block
      mask TypeOptions overflow: Wrap | Saturate | Error
      mask TypeOptions quantization: Truncate | Round  (unbiased: +/- Inf) | Round  (unbiased: even values)
  cvrt3_1_0_imag : Subsystem  AncestorBlock=casper_library_misc/convert_of  mask(convert_of){bit_width_i=17, binary_point_i=14, bit_width_o=17, binary_point_o=14, latency=0, adder_imp=Fabric, overflow=Wrap, quantization=Truncate}
      mask prompts: bit_width_i "Bit Width In"; binary_point_i "Binary Point In"; bit_width_o "Bit Width Out"; binary_point_o "Binary Point Out"; adder_imp "Adder Implementation"; overflow "Overflow Behaviour"; quantization "Quantization Behaviour"
      mask help:
      | Converts from one 2's complement bit-width
      | and/or binary point position to another.
      | Includes underflow/overflow indicator.
      mask init: same as cmult_core/cross_multiplier/cvrt0_0_0_imag
      settings: AttributesFormatString=[17,14]->[17,14]
      mask TypeOptions adder_imp: Fabric | DSP48 | Behavioural | Xilinx Cast Block
      mask TypeOptions overflow: Wrap | Saturate | Error
      mask TypeOptions quantization: Truncate | Round  (unbiased: +/- Inf) | Round  (unbiased: even values)
  cvrt3_1_0_real : Subsystem  AncestorBlock=casper_library_misc/convert_of  mask(convert_of){bit_width_i=17, binary_point_i=14, bit_width_o=17, binary_point_o=14, latency=0, adder_imp=Fabric, overflow=Wrap, quantization=Truncate}
      mask prompts: bit_width_i "Bit Width In"; binary_point_i "Binary Point In"; bit_width_o "Bit Width Out"; binary_point_o "Binary Point Out"; adder_imp "Adder Implementation"; overflow "Overflow Behaviour"; quantization "Quantization Behaviour"
      mask help:
      | Converts from one 2's complement bit-width
      | and/or binary point position to another.
      | Includes underflow/overflow indicator.
      mask init: same as cmult_core/cross_multiplier/cvrt0_0_0_imag
      settings: AttributesFormatString=[17,14]->[17,14]
      mask TypeOptions adder_imp: Fabric | DSP48 | Behavioural | Xilinx Cast Block
      mask TypeOptions overflow: Wrap | Saturate | Error
      mask TypeOptions quantization: Truncate | Round  (unbiased: +/- Inf) | Round  (unbiased: even values)
  cvrt3_2_0_imag : Subsystem  AncestorBlock=casper_library_misc/convert_of  mask(convert_of){bit_width_i=17, binary_point_i=14, bit_width_o=17, binary_point_o=14, latency=0, adder_imp=Fabric, overflow=Wrap, quantization=Truncate}
      mask prompts: bit_width_i "Bit Width In"; binary_point_i "Binary Point In"; bit_width_o "Bit Width Out"; binary_point_o "Binary Point Out"; adder_imp "Adder Implementation"; overflow "Overflow Behaviour"; quantization "Quantization Behaviour"
      mask help:
      | Converts from one 2's complement bit-width
      | and/or binary point position to another.
      | Includes underflow/overflow indicator.
      mask init: same as cmult_core/cross_multiplier/cvrt0_0_0_imag
      settings: AttributesFormatString=[17,14]->[17,14]
      mask TypeOptions adder_imp: Fabric | DSP48 | Behavioural | Xilinx Cast Block
      mask TypeOptions overflow: Wrap | Saturate | Error
      mask TypeOptions quantization: Truncate | Round  (unbiased: +/- Inf) | Round  (unbiased: even values)
  cvrt3_2_0_real : Subsystem  AncestorBlock=casper_library_misc/convert_of  mask(convert_of){bit_width_i=17, binary_point_i=14, bit_width_o=17, binary_point_o=14, latency=0, adder_imp=Fabric, overflow=Wrap, quantization=Truncate}
      mask prompts: bit_width_i "Bit Width In"; binary_point_i "Binary Point In"; bit_width_o "Bit Width Out"; binary_point_o "Binary Point Out"; adder_imp "Adder Implementation"; overflow "Overflow Behaviour"; quantization "Quantization Behaviour"
      mask help:
      | Converts from one 2's complement bit-width
      | and/or binary point position to another.
      | Includes underflow/overflow indicator.
      mask init: same as cmult_core/cross_multiplier/cvrt0_0_0_imag
      settings: AttributesFormatString=[17,14]->[17,14]
      mask TypeOptions adder_imp: Fabric | DSP48 | Behavioural | Xilinx Cast Block
      mask TypeOptions overflow: Wrap | Saturate | Error
      mask TypeOptions quantization: Truncate | Round  (unbiased: +/- Inf) | Round  (unbiased: even values)
  cvrt3_3_0_imag : Subsystem  AncestorBlock=casper_library_misc/convert_of  mask(convert_of){bit_width_i=17, binary_point_i=14, bit_width_o=17, binary_point_o=14, latency=0, adder_imp=Fabric, overflow=Wrap, quantization=Truncate}
      mask prompts: bit_width_i "Bit Width In"; binary_point_i "Binary Point In"; bit_width_o "Bit Width Out"; binary_point_o "Binary Point Out"; adder_imp "Adder Implementation"; overflow "Overflow Behaviour"; quantization "Quantization Behaviour"
      mask help:
      | Converts from one 2's complement bit-width
      | and/or binary point position to another.
      | Includes underflow/overflow indicator.
      mask init: same as cmult_core/cross_multiplier/cvrt0_0_0_imag
      settings: AttributesFormatString=[17,14]->[17,14]
      mask TypeOptions adder_imp: Fabric | DSP48 | Behavioural | Xilinx Cast Block
      mask TypeOptions overflow: Wrap | Saturate | Error
      mask TypeOptions quantization: Truncate | Round  (unbiased: +/- Inf) | Round  (unbiased: even values)
  cvrt3_3_0_real : Subsystem  AncestorBlock=casper_library_misc/convert_of  mask(convert_of){bit_width_i=17, binary_point_i=14, bit_width_o=17, binary_point_o=14, latency=0, adder_imp=Fabric, overflow=Wrap, quantization=Truncate}
      mask prompts: bit_width_i "Bit Width In"; binary_point_i "Binary Point In"; bit_width_o "Bit Width Out"; binary_point_o "Binary Point Out"; adder_imp "Adder Implementation"; overflow "Overflow Behaviour"; quantization "Quantization Behaviour"
      mask help:
      | Converts from one 2's complement bit-width
      | and/or binary point position to another.
      | Includes underflow/overflow indicator.
      mask init: same as cmult_core/cross_multiplier/cvrt0_0_0_imag
      settings: AttributesFormatString=[17,14]->[17,14]
      mask TypeOptions adder_imp: Fabric | DSP48 | Behavioural | Xilinx Cast Block
      mask TypeOptions overflow: Wrap | Saturate | Error
      mask TypeOptions quantization: Truncate | Round  (unbiased: +/- Inf) | Round  (unbiased: even values)
  cvrt3_4_0_imag : Subsystem  AncestorBlock=casper_library_misc/convert_of  mask(convert_of){bit_width_i=17, binary_point_i=14, bit_width_o=17, binary_point_o=14, latency=0, adder_imp=Fabric, overflow=Wrap, quantization=Truncate}
      mask prompts: bit_width_i "Bit Width In"; binary_point_i "Binary Point In"; bit_width_o "Bit Width Out"; binary_point_o "Binary Point Out"; adder_imp "Adder Implementation"; overflow "Overflow Behaviour"; quantization "Quantization Behaviour"
      mask help:
      | Converts from one 2's complement bit-width
      | and/or binary point position to another.
      | Includes underflow/overflow indicator.
      mask init: same as cmult_core/cross_multiplier/cvrt0_0_0_imag
      settings: AttributesFormatString=[17,14]->[17,14]
      mask TypeOptions adder_imp: Fabric | DSP48 | Behavioural | Xilinx Cast Block
      mask TypeOptions overflow: Wrap | Saturate | Error
      mask TypeOptions quantization: Truncate | Round  (unbiased: +/- Inf) | Round  (unbiased: even values)
  cvrt3_4_0_real : Subsystem  AncestorBlock=casper_library_misc/convert_of  mask(convert_of){bit_width_i=17, binary_point_i=14, bit_width_o=17, binary_point_o=14, latency=0, adder_imp=Fabric, overflow=Wrap, quantization=Truncate}
      mask prompts: bit_width_i "Bit Width In"; binary_point_i "Binary Point In"; bit_width_o "Bit Width Out"; binary_point_o "Binary Point Out"; adder_imp "Adder Implementation"; overflow "Overflow Behaviour"; quantization "Quantization Behaviour"
      mask help:
      | Converts from one 2's complement bit-width
      | and/or binary point position to another.
      | Includes underflow/overflow indicator.
      mask init: same as cmult_core/cross_multiplier/cvrt0_0_0_imag
      settings: AttributesFormatString=[17,14]->[17,14]
      mask TypeOptions adder_imp: Fabric | DSP48 | Behavioural | Xilinx Cast Block
      mask TypeOptions overflow: Wrap | Saturate | Error
      mask TypeOptions quantization: Truncate | Round  (unbiased: +/- Inf) | Round  (unbiased: even values)
  cvrt4_0_0_imag : Subsystem  AncestorBlock=casper_library_misc/convert_of  mask(convert_of){bit_width_i=17, binary_point_i=14, bit_width_o=17, binary_point_o=14, latency=0, adder_imp=Fabric, overflow=Wrap, quantization=Truncate}
      mask prompts: bit_width_i "Bit Width In"; binary_point_i "Binary Point In"; bit_width_o "Bit Width Out"; binary_point_o "Binary Point Out"; adder_imp "Adder Implementation"; overflow "Overflow Behaviour"; quantization "Quantization Behaviour"
      mask help:
      | Converts from one 2's complement bit-width
      | and/or binary point position to another.
      | Includes underflow/overflow indicator.
      mask init: same as cmult_core/cross_multiplier/cvrt0_0_0_imag
      settings: AttributesFormatString=[17,14]->[17,14]
      mask TypeOptions adder_imp: Fabric | DSP48 | Behavioural | Xilinx Cast Block
      mask TypeOptions overflow: Wrap | Saturate | Error
      mask TypeOptions quantization: Truncate | Round  (unbiased: +/- Inf) | Round  (unbiased: even values)
  cvrt4_0_0_real : Subsystem  AncestorBlock=casper_library_misc/convert_of  mask(convert_of){bit_width_i=17, binary_point_i=14, bit_width_o=17, binary_point_o=14, latency=0, adder_imp=Fabric, overflow=Wrap, quantization=Truncate}
      mask prompts: bit_width_i "Bit Width In"; binary_point_i "Binary Point In"; bit_width_o "Bit Width Out"; binary_point_o "Binary Point Out"; adder_imp "Adder Implementation"; overflow "Overflow Behaviour"; quantization "Quantization Behaviour"
      mask help:
      | Converts from one 2's complement bit-width
      | and/or binary point position to another.
      | Includes underflow/overflow indicator.
      mask init: same as cmult_core/cross_multiplier/cvrt0_0_0_imag
      settings: AttributesFormatString=[17,14]->[17,14]
      mask TypeOptions adder_imp: Fabric | DSP48 | Behavioural | Xilinx Cast Block
      mask TypeOptions overflow: Wrap | Saturate | Error
      mask TypeOptions quantization: Truncate | Round  (unbiased: +/- Inf) | Round  (unbiased: even values)
  cvrt4_1_0_imag : Subsystem  AncestorBlock=casper_library_misc/convert_of  mask(convert_of){bit_width_i=17, binary_point_i=14, bit_width_o=17, binary_point_o=14, latency=0, adder_imp=Fabric, overflow=Wrap, quantization=Truncate}
      mask prompts: bit_width_i "Bit Width In"; binary_point_i "Binary Point In"; bit_width_o "Bit Width Out"; binary_point_o "Binary Point Out"; adder_imp "Adder Implementation"; overflow "Overflow Behaviour"; quantization "Quantization Behaviour"
      mask help:
      | Converts from one 2's complement bit-width
      | and/or binary point position to another.
      | Includes underflow/overflow indicator.
      mask init: same as cmult_core/cross_multiplier/cvrt0_0_0_imag
      settings: AttributesFormatString=[17,14]->[17,14]
      mask TypeOptions adder_imp: Fabric | DSP48 | Behavioural | Xilinx Cast Block
      mask TypeOptions overflow: Wrap | Saturate | Error
      mask TypeOptions quantization: Truncate | Round  (unbiased: +/- Inf) | Round  (unbiased: even values)
  cvrt4_1_0_real : Subsystem  AncestorBlock=casper_library_misc/convert_of  mask(convert_of){bit_width_i=17, binary_point_i=14, bit_width_o=17, binary_point_o=14, latency=0, adder_imp=Fabric, overflow=Wrap, quantization=Truncate}
      mask prompts: bit_width_i "Bit Width In"; binary_point_i "Binary Point In"; bit_width_o "Bit Width Out"; binary_point_o "Binary Point Out"; adder_imp "Adder Implementation"; overflow "Overflow Behaviour"; quantization "Quantization Behaviour"
      mask help:
      | Converts from one 2's complement bit-width
      | and/or binary point position to another.
      | Includes underflow/overflow indicator.
      mask init: same as cmult_core/cross_multiplier/cvrt0_0_0_imag
      settings: AttributesFormatString=[17,14]->[17,14]
      mask TypeOptions adder_imp: Fabric | DSP48 | Behavioural | Xilinx Cast Block
      mask TypeOptions overflow: Wrap | Saturate | Error
      mask TypeOptions quantization: Truncate | Round  (unbiased: +/- Inf) | Round  (unbiased: even values)
  cvrt4_2_0_imag : Subsystem  AncestorBlock=casper_library_misc/convert_of  mask(convert_of){bit_width_i=17, binary_point_i=14, bit_width_o=17, binary_point_o=14, latency=0, adder_imp=Fabric, overflow=Wrap, quantization=Truncate}
      mask prompts: bit_width_i "Bit Width In"; binary_point_i "Binary Point In"; bit_width_o "Bit Width Out"; binary_point_o "Binary Point Out"; adder_imp "Adder Implementation"; overflow "Overflow Behaviour"; quantization "Quantization Behaviour"
      mask help:
      | Converts from one 2's complement bit-width
      | and/or binary point position to another.
      | Includes underflow/overflow indicator.
      mask init: same as cmult_core/cross_multiplier/cvrt0_0_0_imag
      settings: AttributesFormatString=[17,14]->[17,14]
      mask TypeOptions adder_imp: Fabric | DSP48 | Behavioural | Xilinx Cast Block
      mask TypeOptions overflow: Wrap | Saturate | Error
      mask TypeOptions quantization: Truncate | Round  (unbiased: +/- Inf) | Round  (unbiased: even values)
  cvrt4_2_0_real : Subsystem  AncestorBlock=casper_library_misc/convert_of  mask(convert_of){bit_width_i=17, binary_point_i=14, bit_width_o=17, binary_point_o=14, latency=0, adder_imp=Fabric, overflow=Wrap, quantization=Truncate}
      mask prompts: bit_width_i "Bit Width In"; binary_point_i "Binary Point In"; bit_width_o "Bit Width Out"; binary_point_o "Binary Point Out"; adder_imp "Adder Implementation"; overflow "Overflow Behaviour"; quantization "Quantization Behaviour"
      mask help:
      | Converts from one 2's complement bit-width
      | and/or binary point position to another.
      | Includes underflow/overflow indicator.
      mask init: same as cmult_core/cross_multiplier/cvrt0_0_0_imag
      settings: AttributesFormatString=[17,14]->[17,14]
      mask TypeOptions adder_imp: Fabric | DSP48 | Behavioural | Xilinx Cast Block
      mask TypeOptions overflow: Wrap | Saturate | Error
      mask TypeOptions quantization: Truncate | Round  (unbiased: +/- Inf) | Round  (unbiased: even values)
  cvrt4_3_0_imag : Subsystem  AncestorBlock=casper_library_misc/convert_of  mask(convert_of){bit_width_i=17, binary_point_i=14, bit_width_o=17, binary_point_o=14, latency=0, adder_imp=Fabric, overflow=Wrap, quantization=Truncate}
      mask prompts: bit_width_i "Bit Width In"; binary_point_i "Binary Point In"; bit_width_o "Bit Width Out"; binary_point_o "Binary Point Out"; adder_imp "Adder Implementation"; overflow "Overflow Behaviour"; quantization "Quantization Behaviour"
      mask help:
      | Converts from one 2's complement bit-width
      | and/or binary point position to another.
      | Includes underflow/overflow indicator.
      mask init: same as cmult_core/cross_multiplier/cvrt0_0_0_imag
      settings: AttributesFormatString=[17,14]->[17,14]
      mask TypeOptions adder_imp: Fabric | DSP48 | Behavioural | Xilinx Cast Block
      mask TypeOptions overflow: Wrap | Saturate | Error
      mask TypeOptions quantization: Truncate | Round  (unbiased: +/- Inf) | Round  (unbiased: even values)
  cvrt4_3_0_real : Subsystem  AncestorBlock=casper_library_misc/convert_of  mask(convert_of){bit_width_i=17, binary_point_i=14, bit_width_o=17, binary_point_o=14, latency=0, adder_imp=Fabric, overflow=Wrap, quantization=Truncate}
      mask prompts: bit_width_i "Bit Width In"; binary_point_i "Binary Point In"; bit_width_o "Bit Width Out"; binary_point_o "Binary Point Out"; adder_imp "Adder Implementation"; overflow "Overflow Behaviour"; quantization "Quantization Behaviour"
      mask help:
      | Converts from one 2's complement bit-width
      | and/or binary point position to another.
      | Includes underflow/overflow indicator.
      mask init: same as cmult_core/cross_multiplier/cvrt0_0_0_imag
      settings: AttributesFormatString=[17,14]->[17,14]
      mask TypeOptions adder_imp: Fabric | DSP48 | Behavioural | Xilinx Cast Block
      mask TypeOptions overflow: Wrap | Saturate | Error
      mask TypeOptions quantization: Truncate | Round  (unbiased: +/- Inf) | Round  (unbiased: even values)
  cvrt5_0_0_imag : Subsystem  AncestorBlock=casper_library_misc/convert_of  mask(convert_of){bit_width_i=17, binary_point_i=14, bit_width_o=17, binary_point_o=14, latency=0, adder_imp=Fabric, overflow=Wrap, quantization=Truncate}
      mask prompts: bit_width_i "Bit Width In"; binary_point_i "Binary Point In"; bit_width_o "Bit Width Out"; binary_point_o "Binary Point Out"; adder_imp "Adder Implementation"; overflow "Overflow Behaviour"; quantization "Quantization Behaviour"
      mask help:
      | Converts from one 2's complement bit-width
      | and/or binary point position to another.
      | Includes underflow/overflow indicator.
      mask init: same as cmult_core/cross_multiplier/cvrt0_0_0_imag
      settings: AttributesFormatString=[17,14]->[17,14]
      mask TypeOptions adder_imp: Fabric | DSP48 | Behavioural | Xilinx Cast Block
      mask TypeOptions overflow: Wrap | Saturate | Error
      mask TypeOptions quantization: Truncate | Round  (unbiased: +/- Inf) | Round  (unbiased: even values)
  cvrt5_0_0_real : Subsystem  AncestorBlock=casper_library_misc/convert_of  mask(convert_of){bit_width_i=17, binary_point_i=14, bit_width_o=17, binary_point_o=14, latency=0, adder_imp=Fabric, overflow=Wrap, quantization=Truncate}
      mask prompts: bit_width_i "Bit Width In"; binary_point_i "Binary Point In"; bit_width_o "Bit Width Out"; binary_point_o "Binary Point Out"; adder_imp "Adder Implementation"; overflow "Overflow Behaviour"; quantization "Quantization Behaviour"
      mask help:
      | Converts from one 2's complement bit-width
      | and/or binary point position to another.
      | Includes underflow/overflow indicator.
      mask init: same as cmult_core/cross_multiplier/cvrt0_0_0_imag
      settings: AttributesFormatString=[17,14]->[17,14]
      mask TypeOptions adder_imp: Fabric | DSP48 | Behavioural | Xilinx Cast Block
      mask TypeOptions overflow: Wrap | Saturate | Error
      mask TypeOptions quantization: Truncate | Round  (unbiased: +/- Inf) | Round  (unbiased: even values)
  cvrt5_1_0_imag : Subsystem  AncestorBlock=casper_library_misc/convert_of  mask(convert_of){bit_width_i=17, binary_point_i=14, bit_width_o=17, binary_point_o=14, latency=0, adder_imp=Fabric, overflow=Wrap, quantization=Truncate}
      mask prompts: bit_width_i "Bit Width In"; binary_point_i "Binary Point In"; bit_width_o "Bit Width Out"; binary_point_o "Binary Point Out"; adder_imp "Adder Implementation"; overflow "Overflow Behaviour"; quantization "Quantization Behaviour"
      mask help:
      | Converts from one 2's complement bit-width
      | and/or binary point position to another.
      | Includes underflow/overflow indicator.
      mask init: same as cmult_core/cross_multiplier/cvrt0_0_0_imag
      settings: AttributesFormatString=[17,14]->[17,14]
      mask TypeOptions adder_imp: Fabric | DSP48 | Behavioural | Xilinx Cast Block
      mask TypeOptions overflow: Wrap | Saturate | Error
      mask TypeOptions quantization: Truncate | Round  (unbiased: +/- Inf) | Round  (unbiased: even values)
  cvrt5_1_0_real : Subsystem  AncestorBlock=casper_library_misc/convert_of  mask(convert_of){bit_width_i=17, binary_point_i=14, bit_width_o=17, binary_point_o=14, latency=0, adder_imp=Fabric, overflow=Wrap, quantization=Truncate}
      mask prompts: bit_width_i "Bit Width In"; binary_point_i "Binary Point In"; bit_width_o "Bit Width Out"; binary_point_o "Binary Point Out"; adder_imp "Adder Implementation"; overflow "Overflow Behaviour"; quantization "Quantization Behaviour"
      mask help:
      | Converts from one 2's complement bit-width
      | and/or binary point position to another.
      | Includes underflow/overflow indicator.
      mask init: same as cmult_core/cross_multiplier/cvrt0_0_0_imag
      settings: AttributesFormatString=[17,14]->[17,14]
      mask TypeOptions adder_imp: Fabric | DSP48 | Behavioural | Xilinx Cast Block
      mask TypeOptions overflow: Wrap | Saturate | Error
      mask TypeOptions quantization: Truncate | Round  (unbiased: +/- Inf) | Round  (unbiased: even values)
  cvrt5_2_0_imag : Subsystem  AncestorBlock=casper_library_misc/convert_of  mask(convert_of){bit_width_i=17, binary_point_i=14, bit_width_o=17, binary_point_o=14, latency=0, adder_imp=Fabric, overflow=Wrap, quantization=Truncate}
      mask prompts: bit_width_i "Bit Width In"; binary_point_i "Binary Point In"; bit_width_o "Bit Width Out"; binary_point_o "Binary Point Out"; adder_imp "Adder Implementation"; overflow "Overflow Behaviour"; quantization "Quantization Behaviour"
      mask help:
      | Converts from one 2's complement bit-width
      | and/or binary point position to another.
      | Includes underflow/overflow indicator.
      mask init: same as cmult_core/cross_multiplier/cvrt0_0_0_imag
      settings: AttributesFormatString=[17,14]->[17,14]
      mask TypeOptions adder_imp: Fabric | DSP48 | Behavioural | Xilinx Cast Block
      mask TypeOptions overflow: Wrap | Saturate | Error
      mask TypeOptions quantization: Truncate | Round  (unbiased: +/- Inf) | Round  (unbiased: even values)
  cvrt5_2_0_real : Subsystem  AncestorBlock=casper_library_misc/convert_of  mask(convert_of){bit_width_i=17, binary_point_i=14, bit_width_o=17, binary_point_o=14, latency=0, adder_imp=Fabric, overflow=Wrap, quantization=Truncate}
      mask prompts: bit_width_i "Bit Width In"; binary_point_i "Binary Point In"; bit_width_o "Bit Width Out"; binary_point_o "Binary Point Out"; adder_imp "Adder Implementation"; overflow "Overflow Behaviour"; quantization "Quantization Behaviour"
      mask help:
      | Converts from one 2's complement bit-width
      | and/or binary point position to another.
      | Includes underflow/overflow indicator.
      mask init: same as cmult_core/cross_multiplier/cvrt0_0_0_imag
      settings: AttributesFormatString=[17,14]->[17,14]
      mask TypeOptions adder_imp: Fabric | DSP48 | Behavioural | Xilinx Cast Block
      mask TypeOptions overflow: Wrap | Saturate | Error
      mask TypeOptions quantization: Truncate | Round  (unbiased: +/- Inf) | Round  (unbiased: even values)
  cvrt6_0_0_imag : Subsystem  AncestorBlock=casper_library_misc/convert_of  mask(convert_of){bit_width_i=17, binary_point_i=14, bit_width_o=17, binary_point_o=14, latency=0, adder_imp=Fabric, overflow=Wrap, quantization=Truncate}
      mask prompts: bit_width_i "Bit Width In"; binary_point_i "Binary Point In"; bit_width_o "Bit Width Out"; binary_point_o "Binary Point Out"; adder_imp "Adder Implementation"; overflow "Overflow Behaviour"; quantization "Quantization Behaviour"
      mask help:
      | Converts from one 2's complement bit-width
      | and/or binary point position to another.
      | Includes underflow/overflow indicator.
      mask init: same as cmult_core/cross_multiplier/cvrt0_0_0_imag
      settings: AttributesFormatString=[17,14]->[17,14]
      mask TypeOptions adder_imp: Fabric | DSP48 | Behavioural | Xilinx Cast Block
      mask TypeOptions overflow: Wrap | Saturate | Error
      mask TypeOptions quantization: Truncate | Round  (unbiased: +/- Inf) | Round  (unbiased: even values)
  cvrt6_0_0_real : Subsystem  AncestorBlock=casper_library_misc/convert_of  mask(convert_of){bit_width_i=17, binary_point_i=14, bit_width_o=17, binary_point_o=14, latency=0, adder_imp=Fabric, overflow=Wrap, quantization=Truncate}
      mask prompts: bit_width_i "Bit Width In"; binary_point_i "Binary Point In"; bit_width_o "Bit Width Out"; binary_point_o "Binary Point Out"; adder_imp "Adder Implementation"; overflow "Overflow Behaviour"; quantization "Quantization Behaviour"
      mask help:
      | Converts from one 2's complement bit-width
      | and/or binary point position to another.
      | Includes underflow/overflow indicator.
      mask init: same as cmult_core/cross_multiplier/cvrt0_0_0_imag
      settings: AttributesFormatString=[17,14]->[17,14]
      mask TypeOptions adder_imp: Fabric | DSP48 | Behavioural | Xilinx Cast Block
      mask TypeOptions overflow: Wrap | Saturate | Error
      mask TypeOptions quantization: Truncate | Round  (unbiased: +/- Inf) | Round  (unbiased: even values)
  cvrt6_1_0_imag : Subsystem  AncestorBlock=casper_library_misc/convert_of  mask(convert_of){bit_width_i=17, binary_point_i=14, bit_width_o=17, binary_point_o=14, latency=0, adder_imp=Fabric, overflow=Wrap, quantization=Truncate}
      mask prompts: bit_width_i "Bit Width In"; binary_point_i "Binary Point In"; bit_width_o "Bit Width Out"; binary_point_o "Binary Point Out"; adder_imp "Adder Implementation"; overflow "Overflow Behaviour"; quantization "Quantization Behaviour"
      mask help:
      | Converts from one 2's complement bit-width
      | and/or binary point position to another.
      | Includes underflow/overflow indicator.
      mask init: same as cmult_core/cross_multiplier/cvrt0_0_0_imag
      settings: AttributesFormatString=[17,14]->[17,14]
      mask TypeOptions adder_imp: Fabric | DSP48 | Behavioural | Xilinx Cast Block
      mask TypeOptions overflow: Wrap | Saturate | Error
      mask TypeOptions quantization: Truncate | Round  (unbiased: +/- Inf) | Round  (unbiased: even values)
  cvrt6_1_0_real : Subsystem  AncestorBlock=casper_library_misc/convert_of  mask(convert_of){bit_width_i=17, binary_point_i=14, bit_width_o=17, binary_point_o=14, latency=0, adder_imp=Fabric, overflow=Wrap, quantization=Truncate}
      mask prompts: bit_width_i "Bit Width In"; binary_point_i "Binary Point In"; bit_width_o "Bit Width Out"; binary_point_o "Binary Point Out"; adder_imp "Adder Implementation"; overflow "Overflow Behaviour"; quantization "Quantization Behaviour"
      mask help:
      | Converts from one 2's complement bit-width
      | and/or binary point position to another.
      | Includes underflow/overflow indicator.
      mask init: same as cmult_core/cross_multiplier/cvrt0_0_0_imag
      settings: AttributesFormatString=[17,14]->[17,14]
      mask TypeOptions adder_imp: Fabric | DSP48 | Behavioural | Xilinx Cast Block
      mask TypeOptions overflow: Wrap | Saturate | Error
      mask TypeOptions quantization: Truncate | Round  (unbiased: +/- Inf) | Round  (unbiased: even values)
  cvrt7_0_0_imag : Subsystem  AncestorBlock=casper_library_misc/convert_of  mask(convert_of){bit_width_i=17, binary_point_i=14, bit_width_o=17, binary_point_o=14, latency=0, adder_imp=Fabric, overflow=Wrap, quantization=Truncate}
      mask prompts: bit_width_i "Bit Width In"; binary_point_i "Binary Point In"; bit_width_o "Bit Width Out"; binary_point_o "Binary Point Out"; adder_imp "Adder Implementation"; overflow "Overflow Behaviour"; quantization "Quantization Behaviour"
      mask help:
      | Converts from one 2's complement bit-width
      | and/or binary point position to another.
      | Includes underflow/overflow indicator.
      mask init: same as cmult_core/cross_multiplier/cvrt0_0_0_imag
      settings: AttributesFormatString=[17,14]->[17,14]
      mask TypeOptions adder_imp: Fabric | DSP48 | Behavioural | Xilinx Cast Block
      mask TypeOptions overflow: Wrap | Saturate | Error
      mask TypeOptions quantization: Truncate | Round  (unbiased: +/- Inf) | Round  (unbiased: even values)
  cvrt7_0_0_real : Subsystem  AncestorBlock=casper_library_misc/convert_of  mask(convert_of){bit_width_i=17, binary_point_i=14, bit_width_o=17, binary_point_o=14, latency=0, adder_imp=Fabric, overflow=Wrap, quantization=Truncate}
      mask prompts: bit_width_i "Bit Width In"; binary_point_i "Binary Point In"; bit_width_o "Bit Width Out"; binary_point_o "Binary Point Out"; adder_imp "Adder Implementation"; overflow "Overflow Behaviour"; quantization "Quantization Behaviour"
      mask help:
      | Converts from one 2's complement bit-width
      | and/or binary point position to another.
      | Includes underflow/overflow indicator.
      mask init: same as cmult_core/cross_multiplier/cvrt0_0_0_imag
      settings: AttributesFormatString=[17,14]->[17,14]
      mask TypeOptions adder_imp: Fabric | DSP48 | Behavioural | Xilinx Cast Block
      mask TypeOptions overflow: Wrap | Saturate | Error
      mask TypeOptions quantization: Truncate | Round  (unbiased: +/- Inf) | Round  (unbiased: even values)
  delay0_0_0_{0..3} (4 alike) : xbsIndex_r4/Delay  rst=off  infoeditControl=Selection of Reset will increase slice count due to use of real FFs and instead of SRLs  en=off  latency=1  dbl_ovrd=off  reg_retiming=off  block_type=delay
  delay0_1_0_{0..3} (4 alike) : xbsIndex_r4/Delay  rst=off  infoeditControl=Selection of Reset will increase slice count due to use of real FFs and instead of SRLs  en=off  latency=1  dbl_ovrd=off  reg_retiming=off  block_type=delay
  delay0_2_0_{0..3} (4 alike) : xbsIndex_r4/Delay  rst=off  infoeditControl=Selection of Reset will increase slice count due to use of real FFs and instead of SRLs  en=off  latency=1  dbl_ovrd=off  reg_retiming=off  block_type=delay
  delay0_3_0_{0..3} (4 alike) : xbsIndex_r4/Delay  rst=off  infoeditControl=Selection of Reset will increase slice count due to use of real FFs and instead of SRLs  en=off  latency=1  dbl_ovrd=off  reg_retiming=off  block_type=delay
  delay0_4_0_{0..3} (4 alike) : xbsIndex_r4/Delay  rst=off  infoeditControl=Selection of Reset will increase slice count due to use of real FFs and instead of SRLs  en=off  latency=1  dbl_ovrd=off  reg_retiming=off  block_type=delay
  delay0_5_0_{0..3} (4 alike) : xbsIndex_r4/Delay  rst=off  infoeditControl=Selection of Reset will increase slice count due to use of real FFs and instead of SRLs  en=off  latency=1  dbl_ovrd=off  reg_retiming=off  block_type=delay
  delay0_6_0_{0..3} (4 alike) : xbsIndex_r4/Delay  rst=off  infoeditControl=Selection of Reset will increase slice count due to use of real FFs and instead of SRLs  en=off  latency=1  dbl_ovrd=off  reg_retiming=off  block_type=delay
  delay0_7_0_{0..3} (4 alike) : xbsIndex_r4/Delay  rst=off  infoeditControl=Selection of Reset will increase slice count due to use of real FFs and instead of SRLs  en=off  latency=1  dbl_ovrd=off  reg_retiming=off  block_type=delay
  delay1_0_0_{0..3} (4 alike) : xbsIndex_r4/Delay  rst=off  infoeditControl=Selection of Reset will increase slice count due to use of real FFs and instead of SRLs  en=off  latency=1  dbl_ovrd=off  reg_retiming=off  block_type=delay
  delay1_1_0_{0..3} (4 alike) : xbsIndex_r4/Delay  rst=off  infoeditControl=Selection of Reset will increase slice count due to use of real FFs and instead of SRLs  en=off  latency=1  dbl_ovrd=off  reg_retiming=off  block_type=delay
  delay1_2_0_{0..3} (4 alike) : xbsIndex_r4/Delay  rst=off  infoeditControl=Selection of Reset will increase slice count due to use of real FFs and instead of SRLs  en=off  latency=1  dbl_ovrd=off  reg_retiming=off  block_type=delay
  delay1_3_0_{0..3} (4 alike) : xbsIndex_r4/Delay  rst=off  infoeditControl=Selection of Reset will increase slice count due to use of real FFs and instead of SRLs  en=off  latency=1  dbl_ovrd=off  reg_retiming=off  block_type=delay
  delay1_4_0_{0..3} (4 alike) : xbsIndex_r4/Delay  rst=off  infoeditControl=Selection of Reset will increase slice count due to use of real FFs and instead of SRLs  en=off  latency=1  dbl_ovrd=off  reg_retiming=off  block_type=delay
  delay1_5_0_{0..3} (4 alike) : xbsIndex_r4/Delay  rst=off  infoeditControl=Selection of Reset will increase slice count due to use of real FFs and instead of SRLs  en=off  latency=1  dbl_ovrd=off  reg_retiming=off  block_type=delay
  delay1_6_0_{0..3} (4 alike) : xbsIndex_r4/Delay  rst=off  infoeditControl=Selection of Reset will increase slice count due to use of real FFs and instead of SRLs  en=off  latency=1  dbl_ovrd=off  reg_retiming=off  block_type=delay
  delay2_0_0_{0..3} (4 alike) : xbsIndex_r4/Delay  rst=off  infoeditControl=Selection of Reset will increase slice count due to use of real FFs and instead of SRLs  en=off  latency=1  dbl_ovrd=off  reg_retiming=off  block_type=delay
  delay2_1_0_{0..3} (4 alike) : xbsIndex_r4/Delay  rst=off  infoeditControl=Selection of Reset will increase slice count due to use of real FFs and instead of SRLs  en=off  latency=1  dbl_ovrd=off  reg_retiming=off  block_type=delay
  delay2_2_0_{0..3} (4 alike) : xbsIndex_r4/Delay  rst=off  infoeditControl=Selection of Reset will increase slice count due to use of real FFs and instead of SRLs  en=off  latency=1  dbl_ovrd=off  reg_retiming=off  block_type=delay
  delay2_3_0_{0..3} (4 alike) : xbsIndex_r4/Delay  rst=off  infoeditControl=Selection of Reset will increase slice count due to use of real FFs and instead of SRLs  en=off  latency=1  dbl_ovrd=off  reg_retiming=off  block_type=delay
  delay2_4_0_{0..3} (4 alike) : xbsIndex_r4/Delay  rst=off  infoeditControl=Selection of Reset will increase slice count due to use of real FFs and instead of SRLs  en=off  latency=1  dbl_ovrd=off  reg_retiming=off  block_type=delay
  delay2_5_0_{0..3} (4 alike) : xbsIndex_r4/Delay  rst=off  infoeditControl=Selection of Reset will increase slice count due to use of real FFs and instead of SRLs  en=off  latency=1  dbl_ovrd=off  reg_retiming=off  block_type=delay
  delay3_0_0_{0..3} (4 alike) : xbsIndex_r4/Delay  rst=off  infoeditControl=Selection of Reset will increase slice count due to use of real FFs and instead of SRLs  en=off  latency=1  dbl_ovrd=off  reg_retiming=off  block_type=delay
  delay3_1_0_{0..3} (4 alike) : xbsIndex_r4/Delay  rst=off  infoeditControl=Selection of Reset will increase slice count due to use of real FFs and instead of SRLs  en=off  latency=1  dbl_ovrd=off  reg_retiming=off  block_type=delay
  delay3_2_0_{0..3} (4 alike) : xbsIndex_r4/Delay  rst=off  infoeditControl=Selection of Reset will increase slice count due to use of real FFs and instead of SRLs  en=off  latency=1  dbl_ovrd=off  reg_retiming=off  block_type=delay
  delay3_3_0_{0..3} (4 alike) : xbsIndex_r4/Delay  rst=off  infoeditControl=Selection of Reset will increase slice count due to use of real FFs and instead of SRLs  en=off  latency=1  dbl_ovrd=off  reg_retiming=off  block_type=delay
  delay3_4_0_{0..3} (4 alike) : xbsIndex_r4/Delay  rst=off  infoeditControl=Selection of Reset will increase slice count due to use of real FFs and instead of SRLs  en=off  latency=1  dbl_ovrd=off  reg_retiming=off  block_type=delay
  delay4_0_0_{0..3} (4 alike) : xbsIndex_r4/Delay  rst=off  infoeditControl=Selection of Reset will increase slice count due to use of real FFs and instead of SRLs  en=off  latency=1  dbl_ovrd=off  reg_retiming=off  block_type=delay
  delay4_1_0_{0..3} (4 alike) : xbsIndex_r4/Delay  rst=off  infoeditControl=Selection of Reset will increase slice count due to use of real FFs and instead of SRLs  en=off  latency=1  dbl_ovrd=off  reg_retiming=off  block_type=delay
  delay4_2_0_{0..3} (4 alike) : xbsIndex_r4/Delay  rst=off  infoeditControl=Selection of Reset will increase slice count due to use of real FFs and instead of SRLs  en=off  latency=1  dbl_ovrd=off  reg_retiming=off  block_type=delay
  delay4_3_0_{0..3} (4 alike) : xbsIndex_r4/Delay  rst=off  infoeditControl=Selection of Reset will increase slice count due to use of real FFs and instead of SRLs  en=off  latency=1  dbl_ovrd=off  reg_retiming=off  block_type=delay
  delay5_0_0_{0..3} (4 alike) : xbsIndex_r4/Delay  rst=off  infoeditControl=Selection of Reset will increase slice count due to use of real FFs and instead of SRLs  en=off  latency=1  dbl_ovrd=off  reg_retiming=off  block_type=delay
  delay5_1_0_{0..3} (4 alike) : xbsIndex_r4/Delay  rst=off  infoeditControl=Selection of Reset will increase slice count due to use of real FFs and instead of SRLs  en=off  latency=1  dbl_ovrd=off  reg_retiming=off  block_type=delay
  delay5_2_0_{0..3} (4 alike) : xbsIndex_r4/Delay  rst=off  infoeditControl=Selection of Reset will increase slice count due to use of real FFs and instead of SRLs  en=off  latency=1  dbl_ovrd=off  reg_retiming=off  block_type=delay
  delay6_0_0_{0..3} (4 alike) : xbsIndex_r4/Delay  rst=off  infoeditControl=Selection of Reset will increase slice count due to use of real FFs and instead of SRLs  en=off  latency=1  dbl_ovrd=off  reg_retiming=off  block_type=delay
  delay6_1_0_{0..3} (4 alike) : xbsIndex_r4/Delay  rst=off  infoeditControl=Selection of Reset will increase slice count due to use of real FFs and instead of SRLs  en=off  latency=1  dbl_ovrd=off  reg_retiming=off  block_type=delay
  delay7_0_0_{0..3} (4 alike) : xbsIndex_r4/Delay  rst=off  infoeditControl=Selection of Reset will increase slice count due to use of real FFs and instead of SRLs  en=off  latency=1  dbl_ovrd=off  reg_retiming=off  block_type=delay
  pack0_0 : Subsystem  AncestorBlock=casper_library_flow_control/bus_create  mask(bus_create){inputNum=aggregation}
      mask prompts: inputNum "Number of inputs:"
      mask init:
      | bus_create_init(gcb,...
      |     'inputNum', inputNum);
  pack0_1 : Subsystem  AncestorBlock=casper_library_flow_control/bus_create  mask(bus_create){inputNum=aggregation}
      mask prompts: inputNum "Number of inputs:"
      mask init:
      | bus_create_init(gcb,...
      |     'inputNum', inputNum);
  pack0_2 : Subsystem  AncestorBlock=casper_library_flow_control/bus_create  mask(bus_create){inputNum=aggregation}
      mask prompts: inputNum "Number of inputs:"
      mask init:
      | bus_create_init(gcb,...
      |     'inputNum', inputNum);
  pack0_3 : Subsystem  AncestorBlock=casper_library_flow_control/bus_create  mask(bus_create){inputNum=aggregation}
      mask prompts: inputNum "Number of inputs:"
      mask init:
      | bus_create_init(gcb,...
      |     'inputNum', inputNum);
  pack0_4 : Subsystem  AncestorBlock=casper_library_flow_control/bus_create  mask(bus_create){inputNum=aggregation}
      mask prompts: inputNum "Number of inputs:"
      mask init:
      | bus_create_init(gcb,...
      |     'inputNum', inputNum);
  pack0_5 : Subsystem  AncestorBlock=casper_library_flow_control/bus_create  mask(bus_create){inputNum=aggregation}
      mask prompts: inputNum "Number of inputs:"
      mask init:
      | bus_create_init(gcb,...
      |     'inputNum', inputNum);
  pack0_6 : Subsystem  AncestorBlock=casper_library_flow_control/bus_create  mask(bus_create){inputNum=aggregation}
      mask prompts: inputNum "Number of inputs:"
      mask init:
      | bus_create_init(gcb,...
      |     'inputNum', inputNum);
  pack0_7 : Subsystem  AncestorBlock=casper_library_flow_control/bus_create  mask(bus_create){inputNum=aggregation}
      mask prompts: inputNum "Number of inputs:"
      mask init:
      | bus_create_init(gcb,...
      |     'inputNum', inputNum);
  pack1_0 : Subsystem  AncestorBlock=casper_library_flow_control/bus_create  mask(bus_create){inputNum=aggregation}
      mask prompts: inputNum "Number of inputs:"
      mask init:
      | bus_create_init(gcb,...
      |     'inputNum', inputNum);
  pack1_1 : Subsystem  AncestorBlock=casper_library_flow_control/bus_create  mask(bus_create){inputNum=aggregation}
      mask prompts: inputNum "Number of inputs:"
      mask init:
      | bus_create_init(gcb,...
      |     'inputNum', inputNum);
  pack1_2 : Subsystem  AncestorBlock=casper_library_flow_control/bus_create  mask(bus_create){inputNum=aggregation}
      mask prompts: inputNum "Number of inputs:"
      mask init:
      | bus_create_init(gcb,...
      |     'inputNum', inputNum);
  pack1_3 : Subsystem  AncestorBlock=casper_library_flow_control/bus_create  mask(bus_create){inputNum=aggregation}
      mask prompts: inputNum "Number of inputs:"
      mask init:
      | bus_create_init(gcb,...
      |     'inputNum', inputNum);
  pack1_4 : Subsystem  AncestorBlock=casper_library_flow_control/bus_create  mask(bus_create){inputNum=aggregation}
      mask prompts: inputNum "Number of inputs:"
      mask init:
      | bus_create_init(gcb,...
      |     'inputNum', inputNum);
  pack1_5 : Subsystem  AncestorBlock=casper_library_flow_control/bus_create  mask(bus_create){inputNum=aggregation}
      mask prompts: inputNum "Number of inputs:"
      mask init:
      | bus_create_init(gcb,...
      |     'inputNum', inputNum);
  pack1_6 : Subsystem  AncestorBlock=casper_library_flow_control/bus_create  mask(bus_create){inputNum=aggregation}
      mask prompts: inputNum "Number of inputs:"
      mask init:
      | bus_create_init(gcb,...
      |     'inputNum', inputNum);
  pack2_0 : Subsystem  AncestorBlock=casper_library_flow_control/bus_create  mask(bus_create){inputNum=aggregation}
      mask prompts: inputNum "Number of inputs:"
      mask init:
      | bus_create_init(gcb,...
      |     'inputNum', inputNum);
  pack2_1 : Subsystem  AncestorBlock=casper_library_flow_control/bus_create  mask(bus_create){inputNum=aggregation}
      mask prompts: inputNum "Number of inputs:"
      mask init:
      | bus_create_init(gcb,...
      |     'inputNum', inputNum);
  pack2_2 : Subsystem  AncestorBlock=casper_library_flow_control/bus_create  mask(bus_create){inputNum=aggregation}
      mask prompts: inputNum "Number of inputs:"
      mask init:
      | bus_create_init(gcb,...
      |     'inputNum', inputNum);
  pack2_3 : Subsystem  AncestorBlock=casper_library_flow_control/bus_create  mask(bus_create){inputNum=aggregation}
      mask prompts: inputNum "Number of inputs:"
      mask init:
      | bus_create_init(gcb,...
      |     'inputNum', inputNum);
  pack2_4 : Subsystem  AncestorBlock=casper_library_flow_control/bus_create  mask(bus_create){inputNum=aggregation}
      mask prompts: inputNum "Number of inputs:"
      mask init:
      | bus_create_init(gcb,...
      |     'inputNum', inputNum);
  pack2_5 : Subsystem  AncestorBlock=casper_library_flow_control/bus_create  mask(bus_create){inputNum=aggregation}
      mask prompts: inputNum "Number of inputs:"
      mask init:
      | bus_create_init(gcb,...
      |     'inputNum', inputNum);
  pack3_0 : Subsystem  AncestorBlock=casper_library_flow_control/bus_create  mask(bus_create){inputNum=aggregation}
      mask prompts: inputNum "Number of inputs:"
      mask init:
      | bus_create_init(gcb,...
      |     'inputNum', inputNum);
  pack3_1 : Subsystem  AncestorBlock=casper_library_flow_control/bus_create  mask(bus_create){inputNum=aggregation}
      mask prompts: inputNum "Number of inputs:"
      mask init:
      | bus_create_init(gcb,...
      |     'inputNum', inputNum);
  pack3_2 : Subsystem  AncestorBlock=casper_library_flow_control/bus_create  mask(bus_create){inputNum=aggregation}
      mask prompts: inputNum "Number of inputs:"
      mask init:
      | bus_create_init(gcb,...
      |     'inputNum', inputNum);
  pack3_3 : Subsystem  AncestorBlock=casper_library_flow_control/bus_create  mask(bus_create){inputNum=aggregation}
      mask prompts: inputNum "Number of inputs:"
      mask init:
      | bus_create_init(gcb,...
      |     'inputNum', inputNum);
  pack3_4 : Subsystem  AncestorBlock=casper_library_flow_control/bus_create  mask(bus_create){inputNum=aggregation}
      mask prompts: inputNum "Number of inputs:"
      mask init:
      | bus_create_init(gcb,...
      |     'inputNum', inputNum);
  pack4_0 : Subsystem  AncestorBlock=casper_library_flow_control/bus_create  mask(bus_create){inputNum=aggregation}
      mask prompts: inputNum "Number of inputs:"
      mask init:
      | bus_create_init(gcb,...
      |     'inputNum', inputNum);
  pack4_1 : Subsystem  AncestorBlock=casper_library_flow_control/bus_create  mask(bus_create){inputNum=aggregation}
      mask prompts: inputNum "Number of inputs:"
      mask init:
      | bus_create_init(gcb,...
      |     'inputNum', inputNum);
  pack4_2 : Subsystem  AncestorBlock=casper_library_flow_control/bus_create  mask(bus_create){inputNum=aggregation}
      mask prompts: inputNum "Number of inputs:"
      mask init:
      | bus_create_init(gcb,...
      |     'inputNum', inputNum);
  pack4_3 : Subsystem  AncestorBlock=casper_library_flow_control/bus_create  mask(bus_create){inputNum=aggregation}
      mask prompts: inputNum "Number of inputs:"
      mask init:
      | bus_create_init(gcb,...
      |     'inputNum', inputNum);
  pack5_0 : Subsystem  AncestorBlock=casper_library_flow_control/bus_create  mask(bus_create){inputNum=aggregation}
      mask prompts: inputNum "Number of inputs:"
      mask init:
      | bus_create_init(gcb,...
      |     'inputNum', inputNum);
  pack5_1 : Subsystem  AncestorBlock=casper_library_flow_control/bus_create  mask(bus_create){inputNum=aggregation}
      mask prompts: inputNum "Number of inputs:"
      mask init:
      | bus_create_init(gcb,...
      |     'inputNum', inputNum);
  pack5_2 : Subsystem  AncestorBlock=casper_library_flow_control/bus_create  mask(bus_create){inputNum=aggregation}
      mask prompts: inputNum "Number of inputs:"
      mask init:
      | bus_create_init(gcb,...
      |     'inputNum', inputNum);
  pack6_0 : Subsystem  AncestorBlock=casper_library_flow_control/bus_create  mask(bus_create){inputNum=aggregation}
      mask prompts: inputNum "Number of inputs:"
      mask init:
      | bus_create_init(gcb,...
      |     'inputNum', inputNum);
  pack6_1 : Subsystem  AncestorBlock=casper_library_flow_control/bus_create  mask(bus_create){inputNum=aggregation}
      mask prompts: inputNum "Number of inputs:"
      mask init:
      | bus_create_init(gcb,...
      |     'inputNum', inputNum);
  pack7_0 : Subsystem  AncestorBlock=casper_library_flow_control/bus_create  mask(bus_create){inputNum=aggregation}
      mask prompts: inputNum "Number of inputs:"
      mask init:
      | bus_create_init(gcb,...
      |     'inputNum', inputNum);
  ri_to_c0_0_0 : casper_library_misc/ri_to_c
  ri_to_c0_1_0 : casper_library_misc/ri_to_c
  ri_to_c0_2_0 : casper_library_misc/ri_to_c
  ri_to_c0_3_0 : casper_library_misc/ri_to_c
  ri_to_c0_4_0 : casper_library_misc/ri_to_c
  ri_to_c0_5_0 : casper_library_misc/ri_to_c
  ri_to_c0_6_0 : casper_library_misc/ri_to_c
  ri_to_c0_7_0 : casper_library_misc/ri_to_c
  ri_to_c1_0_0 : casper_library_misc/ri_to_c
  ri_to_c1_1_0 : casper_library_misc/ri_to_c
  ri_to_c1_2_0 : casper_library_misc/ri_to_c
  ri_to_c1_3_0 : casper_library_misc/ri_to_c
  ri_to_c1_4_0 : casper_library_misc/ri_to_c
  ri_to_c1_5_0 : casper_library_misc/ri_to_c
  ri_to_c1_6_0 : casper_library_misc/ri_to_c
  ri_to_c2_0_0 : casper_library_misc/ri_to_c
  ri_to_c2_1_0 : casper_library_misc/ri_to_c
  ri_to_c2_2_0 : casper_library_misc/ri_to_c
  ri_to_c2_3_0 : casper_library_misc/ri_to_c
  ri_to_c2_4_0 : casper_library_misc/ri_to_c
  ri_to_c2_5_0 : casper_library_misc/ri_to_c
  ri_to_c3_0_0 : casper_library_misc/ri_to_c
  ri_to_c3_1_0 : casper_library_misc/ri_to_c
  ri_to_c3_2_0 : casper_library_misc/ri_to_c
  ri_to_c3_3_0 : casper_library_misc/ri_to_c
  ri_to_c3_4_0 : casper_library_misc/ri_to_c
  ri_to_c4_0_0 : casper_library_misc/ri_to_c
  ri_to_c4_1_0 : casper_library_misc/ri_to_c
  ri_to_c4_2_0 : casper_library_misc/ri_to_c
  ri_to_c4_3_0 : casper_library_misc/ri_to_c
  ri_to_c5_0_0 : casper_library_misc/ri_to_c
  ri_to_c5_1_0 : casper_library_misc/ri_to_c
  ri_to_c5_2_0 : casper_library_misc/ri_to_c
  ri_to_c6_0_0 : casper_library_misc/ri_to_c
  ri_to_c6_1_0 : casper_library_misc/ri_to_c
  ri_to_c7_0_0 : casper_library_misc/ri_to_c
  sync_delay : xbsIndex_r4/Delay  rst=off  infoeditControl=Selection of Reset will increase slice count due to use of real FFs and instead of SRLs  en=off  latency=mult_latency+add_latency+1+conv_latency  dbl_ovrd=off  reg_retiming=off  block_type=delay
  unpack0 : Subsystem  AncestorBlock=casper_library_flow_control/bus_expand  mask(bus_expand){mode=divisions of equal size, outputNum=aggregation, outputWidth=bit_width_in*2, outputBinaryPt=0, outputArithmeticType=0, show_format=off, outputToWorkspace=off, variablePrefix=out, outputToModelAsWell=on}
      mask prompts: outputNum "Number of outputs:"; outputWidth "Output width:"; outputBinaryPt "Output binary point position:"; outputArithmeticType "Output arithmetic type (ufix=0, fix=1, bool=2):"; show_format "Print format string?"; outputToWorkspace "Output to workspace?"; variablePrefix "Variable name prefix:"; outputToModelAsWell "Output to model as well?"
      mask help:
      | Expands a 'bus' made using a bus_create or Xilinx
      | concat block.
      | The input will be divided into the specified number
      | of outputs with the specified arithmetic types.
      | Divisions are made from most significant bit.
      mask init:
      | bus_expand_init(gcb,...
      |     'mode', mode, ...
      |     'outputNum', outputNum, ...
      |     'outputWidth', outputWidth, ...
      |     'outputBinaryPt', outputBinaryPt, ...
      |     'outputArithmeticType', outputArithmeticType, ...
      |     'show_format', show_format, ...
      |     'outputToWorkspace', outputToWorkspace, ...
      |     'variablePrefix', variablePrefix, ...
      |     'outputToModelAsWell', outputToModelAsWell);
      settings: AttributesFormatString=1 outputs
      mask TypeOptions mode: divisions of equal size | divisions of arbitrary size
      mask Callback mode: bus_expand_callback();
      mask Callback outputWidth: bus_expand_callback();
      mask Callback outputToWorkspace: bus_expand_callback();
  unpack1 : Subsystem  AncestorBlock=casper_library_flow_control/bus_expand  mask(bus_expand){mode=divisions of equal size, outputNum=aggregation, outputWidth=bit_width_in*2, outputBinaryPt=0, outputArithmeticType=0, show_format=off, outputToWorkspace=off, variablePrefix=out, outputToModelAsWell=on}
      mask prompts: outputNum "Number of outputs:"; outputWidth "Output width:"; outputBinaryPt "Output binary point position:"; outputArithmeticType "Output arithmetic type (ufix=0, fix=1, bool=2):"; show_format "Print format string?"; outputToWorkspace "Output to workspace?"; variablePrefix "Variable name prefix:"; outputToModelAsWell "Output to model as well?"
      mask help:
      | Expands a 'bus' made using a bus_create or Xilinx
      | concat block.
      | The input will be divided into the specified number
      | of outputs with the specified arithmetic types.
      | Divisions are made from most significant bit.
      mask init: same as cmult_core/cross_multiplier/unpack0
      settings: AttributesFormatString=1 outputs
      mask TypeOptions mode: divisions of equal size | divisions of arbitrary size
      mask Callback mode: bus_expand_callback();
      mask Callback outputWidth: bus_expand_callback();
      mask Callback outputToWorkspace: bus_expand_callback();
  unpack2 : Subsystem  AncestorBlock=casper_library_flow_control/bus_expand  mask(bus_expand){mode=divisions of equal size, outputNum=aggregation, outputWidth=bit_width_in*2, outputBinaryPt=0, outputArithmeticType=0, show_format=off, outputToWorkspace=off, variablePrefix=out, outputToModelAsWell=on}
      mask prompts: outputNum "Number of outputs:"; outputWidth "Output width:"; outputBinaryPt "Output binary point position:"; outputArithmeticType "Output arithmetic type (ufix=0, fix=1, bool=2):"; show_format "Print format string?"; outputToWorkspace "Output to workspace?"; variablePrefix "Variable name prefix:"; outputToModelAsWell "Output to model as well?"
      mask help:
      | Expands a 'bus' made using a bus_create or Xilinx
      | concat block.
      | The input will be divided into the specified number
      | of outputs with the specified arithmetic types.
      | Divisions are made from most significant bit.
      mask init: same as cmult_core/cross_multiplier/unpack0
      settings: AttributesFormatString=1 outputs
      mask TypeOptions mode: divisions of equal size | divisions of arbitrary size
      mask Callback mode: bus_expand_callback();
      mask Callback outputWidth: bus_expand_callback();
      mask Callback outputToWorkspace: bus_expand_callback();
  unpack3 : Subsystem  AncestorBlock=casper_library_flow_control/bus_expand  mask(bus_expand){mode=divisions of equal size, outputNum=aggregation, outputWidth=bit_width_in*2, outputBinaryPt=0, outputArithmeticType=0, show_format=off, outputToWorkspace=off, variablePrefix=out, outputToModelAsWell=on}
      mask prompts: outputNum "Number of outputs:"; outputWidth "Output width:"; outputBinaryPt "Output binary point position:"; outputArithmeticType "Output arithmetic type (ufix=0, fix=1, bool=2):"; show_format "Print format string?"; outputToWorkspace "Output to workspace?"; variablePrefix "Variable name prefix:"; outputToModelAsWell "Output to model as well?"
      mask help:
      | Expands a 'bus' made using a bus_create or Xilinx
      | concat block.
      | The input will be divided into the specified number
      | of outputs with the specified arithmetic types.
      | Divisions are made from most significant bit.
      mask init: same as cmult_core/cross_multiplier/unpack0
      settings: AttributesFormatString=1 outputs
      mask TypeOptions mode: divisions of equal size | divisions of arbitrary size
      mask Callback mode: bus_expand_callback();
      mask Callback outputWidth: bus_expand_callback();
      mask Callback outputToWorkspace: bus_expand_callback();
  unpack4 : Subsystem  AncestorBlock=casper_library_flow_control/bus_expand  mask(bus_expand){mode=divisions of equal size, outputNum=aggregation, outputWidth=bit_width_in*2, outputBinaryPt=0, outputArithmeticType=0, show_format=off, outputToWorkspace=off, variablePrefix=out, outputToModelAsWell=on}
      mask prompts: outputNum "Number of outputs:"; outputWidth "Output width:"; outputBinaryPt "Output binary point position:"; outputArithmeticType "Output arithmetic type (ufix=0, fix=1, bool=2):"; show_format "Print format string?"; outputToWorkspace "Output to workspace?"; variablePrefix "Variable name prefix:"; outputToModelAsWell "Output to model as well?"
      mask help:
      | Expands a 'bus' made using a bus_create or Xilinx
      | concat block.
      | The input will be divided into the specified number
      | of outputs with the specified arithmetic types.
      | Divisions are made from most significant bit.
      mask init: same as cmult_core/cross_multiplier/unpack0
      settings: AttributesFormatString=1 outputs
      mask TypeOptions mode: divisions of equal size | divisions of arbitrary size
      mask Callback mode: bus_expand_callback();
      mask Callback outputWidth: bus_expand_callback();
      mask Callback outputToWorkspace: bus_expand_callback();
  unpack5 : Subsystem  AncestorBlock=casper_library_flow_control/bus_expand  mask(bus_expand){mode=divisions of equal size, outputNum=aggregation, outputWidth=bit_width_in*2, outputBinaryPt=0, outputArithmeticType=0, show_format=off, outputToWorkspace=off, variablePrefix=out, outputToModelAsWell=on}
      mask prompts: outputNum "Number of outputs:"; outputWidth "Output width:"; outputBinaryPt "Output binary point position:"; outputArithmeticType "Output arithmetic type (ufix=0, fix=1, bool=2):"; show_format "Print format string?"; outputToWorkspace "Output to workspace?"; variablePrefix "Variable name prefix:"; outputToModelAsWell "Output to model as well?"
      mask help:
      | Expands a 'bus' made using a bus_create or Xilinx
      | concat block.
      | The input will be divided into the specified number
      | of outputs with the specified arithmetic types.
      | Divisions are made from most significant bit.
      mask init: same as cmult_core/cross_multiplier/unpack0
      settings: AttributesFormatString=1 outputs
      mask TypeOptions mode: divisions of equal size | divisions of arbitrary size
      mask Callback mode: bus_expand_callback();
      mask Callback outputWidth: bus_expand_callback();
      mask Callback outputToWorkspace: bus_expand_callback();
  unpack6 : Subsystem  AncestorBlock=casper_library_flow_control/bus_expand  mask(bus_expand){mode=divisions of equal size, outputNum=aggregation, outputWidth=bit_width_in*2, outputBinaryPt=0, outputArithmeticType=0, show_format=off, outputToWorkspace=off, variablePrefix=out, outputToModelAsWell=on}
      mask prompts: outputNum "Number of outputs:"; outputWidth "Output width:"; outputBinaryPt "Output binary point position:"; outputArithmeticType "Output arithmetic type (ufix=0, fix=1, bool=2):"; show_format "Print format string?"; outputToWorkspace "Output to workspace?"; variablePrefix "Variable name prefix:"; outputToModelAsWell "Output to model as well?"
      mask help:
      | Expands a 'bus' made using a bus_create or Xilinx
      | concat block.
      | The input will be divided into the specified number
      | of outputs with the specified arithmetic types.
      | Divisions are made from most significant bit.
      mask init: same as cmult_core/cross_multiplier/unpack0
      settings: AttributesFormatString=1 outputs
      mask TypeOptions mode: divisions of equal size | divisions of arbitrary size
      mask Callback mode: bus_expand_callback();
      mask Callback outputWidth: bus_expand_callback();
      mask Callback outputToWorkspace: bus_expand_callback();
  unpack7 : Subsystem  AncestorBlock=casper_library_flow_control/bus_expand  mask(bus_expand){mode=divisions of equal size, outputNum=aggregation, outputWidth=bit_width_in*2, outputBinaryPt=0, outputArithmeticType=0, show_format=off, outputToWorkspace=off, variablePrefix=out, outputToModelAsWell=on}
      mask prompts: outputNum "Number of outputs:"; outputWidth "Output width:"; outputBinaryPt "Output binary point position:"; outputArithmeticType "Output arithmetic type (ufix=0, fix=1, bool=2):"; show_format "Print format string?"; outputToWorkspace "Output to workspace?"; variablePrefix "Variable name prefix:"; outputToModelAsWell "Output to model as well?"
      mask help:
      | Expands a 'bus' made using a bus_create or Xilinx
      | concat block.
      | The input will be divided into the specified number
      | of outputs with the specified arithmetic types.
      | Divisions are made from most significant bit.
      mask init: same as cmult_core/cross_multiplier/unpack0
      settings: AttributesFormatString=1 outputs
      mask TypeOptions mode: divisions of equal size | divisions of arbitrary size
      mask Callback mode: bus_expand_callback();
      mask Callback outputWidth: bus_expand_callback();
      mask Callback outputToWorkspace: bus_expand_callback();
  sync_out : Outport
  din0_x_din0* : Outport  Port=2
  din0_x_din1* : Outport  Port=3
  din0_x_din2* : Outport  Port=4
  din0_x_din3* : Outport  Port=5
  din0_x_din4* : Outport  Port=6
  din0_x_din5* : Outport  Port=7
  din0_x_din6* : Outport  Port=8
  din0_x_din7* : Outport  Port=9
  din1_x_din1* : Outport  Port=10
  din1_x_din2* : Outport  Port=11
  din1_x_din3* : Outport  Port=12
  din1_x_din4* : Outport  Port=13
  din1_x_din5* : Outport  Port=14
  din1_x_din6* : Outport  Port=15
  din1_x_din7* : Outport  Port=16
  din2_x_din2* : Outport  Port=17
  din2_x_din3* : Outport  Port=18
  din2_x_din4* : Outport  Port=19
  din2_x_din5* : Outport  Port=20
  din2_x_din6* : Outport  Port=21
  din2_x_din7* : Outport  Port=22
  din3_x_din3* : Outport  Port=23
  din3_x_din4* : Outport  Port=24
  din3_x_din5* : Outport  Port=25
  din3_x_din6* : Outport  Port=26
  din3_x_din7* : Outport  Port=27
  din4_x_din4* : Outport  Port=28
  din4_x_din5* : Outport  Port=29
  din4_x_din6* : Outport  Port=30
  din4_x_din7* : Outport  Port=31
  din5_x_din5* : Outport  Port=32
  din5_x_din6* : Outport  Port=33
  din5_x_din7* : Outport  Port=34
  din6_x_din6* : Outport  Port=35
  din6_x_din7* : Outport  Port=36
  din7_x_din7* : Outport  Port=37
  wires:
  sync_in/1 -> sync_delay/1
  sync_delay/1 -> sync_out/1
  din0/1 -> unpack0/1(bus_in)
  unpack0/1(msb_lsb_out1) -> c_to_ri0_0/1
  din1/1 -> unpack1/1(bus_in)
  unpack1/1(msb_lsb_out1) -> c_to_ri1_0/1
  din2/1 -> unpack2/1(bus_in)
  unpack2/1(msb_lsb_out1) -> c_to_ri2_0/1
  din3/1 -> unpack3/1(bus_in)
  unpack3/1(msb_lsb_out1) -> c_to_ri3_0/1
  din4/1 -> unpack4/1(bus_in)
  unpack4/1(msb_lsb_out1) -> c_to_ri4_0/1
  din5/1 -> unpack5/1(bus_in)
  unpack5/1(msb_lsb_out1) -> c_to_ri5_0/1
  din6/1 -> unpack6/1(bus_in)
  unpack6/1(msb_lsb_out1) -> c_to_ri6_0/1
  din7/1 -> unpack7/1(bus_in)
  unpack7/1(msb_lsb_out1) -> c_to_ri7_0/1
  c_to_ri0_0/1 -> delay0_0_0_0/1, delay0_0_0_2/1, delay0_1_0_0/1, delay0_2_0_0/1, delay0_3_0_0/1, delay0_4_0_0/1, delay0_5_0_0/1, delay0_6_0_0/1, delay0_7_0_0/1
  delay0_0_0_0/1 -> cmult0_0_0/1
  c_to_ri0_0/2 -> delay0_0_0_1/1, delay0_0_0_3/1, delay0_1_0_1/1, delay0_2_0_1/1, delay0_3_0_1/1, delay0_4_0_1/1, delay0_5_0_1/1, delay0_6_0_1/1, delay0_7_0_1/1
  delay0_0_0_1/1 -> cmult0_0_0/2
  delay0_0_0_2/1 -> cmult0_0_0/3
  delay0_0_0_3/1 -> cmult0_0_0/4
  cmult0_0_0/1 -> cvrt0_0_0_real/1(din)
  cmult0_0_0/2 -> cvrt0_0_0_imag/1(din)
  cvrt0_0_0_real/1(dout) -> ri_to_c0_0_0/1
  cvrt0_0_0_imag/1(dout) -> ri_to_c0_0_0/2
  ri_to_c0_0_0/1 -> pack0_0/1(in1)
  pack0_0/1(bus_out) -> din0_x_din0*/1
  delay0_1_0_0/1 -> cmult0_1_0/1
  delay0_1_0_1/1 -> cmult0_1_0/2
  c_to_ri1_0/1 -> delay0_1_0_2/1, delay1_0_0_0/1, delay1_0_0_2/1, delay1_1_0_0/1, delay1_2_0_0/1, delay1_3_0_0/1, delay1_4_0_0/1, delay1_5_0_0/1, delay1_6_0_0/1
  delay0_1_0_2/1 -> cmult0_1_0/3
  c_to_ri1_0/2 -> delay0_1_0_3/1, delay1_0_0_1/1, delay1_0_0_3/1, delay1_1_0_1/1, delay1_2_0_1/1, delay1_3_0_1/1, delay1_4_0_1/1, delay1_5_0_1/1, delay1_6_0_1/1
  delay0_1_0_3/1 -> cmult0_1_0/4
  cmult0_1_0/1 -> cvrt0_1_0_real/1(din)
  cmult0_1_0/2 -> cvrt0_1_0_imag/1(din)
  cvrt0_1_0_real/1(dout) -> ri_to_c0_1_0/1
  cvrt0_1_0_imag/1(dout) -> ri_to_c0_1_0/2
  ri_to_c0_1_0/1 -> pack0_1/1(in1)
  pack0_1/1(bus_out) -> din0_x_din1*/1
  delay0_2_0_0/1 -> cmult0_2_0/1
  delay0_2_0_1/1 -> cmult0_2_0/2
  c_to_ri2_0/1 -> delay0_2_0_2/1, delay1_1_0_2/1, delay2_0_0_0/1, delay2_0_0_2/1, delay2_1_0_0/1, delay2_2_0_0/1, delay2_3_0_0/1, delay2_4_0_0/1, delay2_5_0_0/1
  delay0_2_0_2/1 -> cmult0_2_0/3
  c_to_ri2_0/2 -> delay0_2_0_3/1, delay1_1_0_3/1, delay2_0_0_1/1, delay2_0_0_3/1, delay2_1_0_1/1, delay2_2_0_1/1, delay2_3_0_1/1, delay2_4_0_1/1, delay2_5_0_1/1
  delay0_2_0_3/1 -> cmult0_2_0/4
  cmult0_2_0/1 -> cvrt0_2_0_real/1(din)
  cmult0_2_0/2 -> cvrt0_2_0_imag/1(din)
  cvrt0_2_0_real/1(dout) -> ri_to_c0_2_0/1
  cvrt0_2_0_imag/1(dout) -> ri_to_c0_2_0/2
  ri_to_c0_2_0/1 -> pack0_2/1(in1)
  pack0_2/1(bus_out) -> din0_x_din2*/1
  delay0_3_0_0/1 -> cmult0_3_0/1
  delay0_3_0_1/1 -> cmult0_3_0/2
  c_to_ri3_0/1 -> delay0_3_0_2/1, delay1_2_0_2/1, delay2_1_0_2/1, delay3_0_0_0/1, delay3_0_0_2/1, delay3_1_0_0/1, delay3_2_0_0/1, delay3_3_0_0/1, delay3_4_0_0/1
  delay0_3_0_2/1 -> cmult0_3_0/3
  c_to_ri3_0/2 -> delay0_3_0_3/1, delay1_2_0_3/1, delay2_1_0_3/1, delay3_0_0_1/1, delay3_0_0_3/1, delay3_1_0_1/1, delay3_2_0_1/1, delay3_3_0_1/1, delay3_4_0_1/1
  delay0_3_0_3/1 -> cmult0_3_0/4
  cmult0_3_0/1 -> cvrt0_3_0_real/1(din)
  cmult0_3_0/2 -> cvrt0_3_0_imag/1(din)
  cvrt0_3_0_real/1(dout) -> ri_to_c0_3_0/1
  cvrt0_3_0_imag/1(dout) -> ri_to_c0_3_0/2
  ri_to_c0_3_0/1 -> pack0_3/1(in1)
  pack0_3/1(bus_out) -> din0_x_din3*/1
  delay0_4_0_0/1 -> cmult0_4_0/1
  delay0_4_0_1/1 -> cmult0_4_0/2
  c_to_ri4_0/1 -> delay0_4_0_2/1, delay1_3_0_2/1, delay2_2_0_2/1, delay3_1_0_2/1, delay4_0_0_0/1, delay4_0_0_2/1, delay4_1_0_0/1, delay4_2_0_0/1, delay4_3_0_0/1
  delay0_4_0_2/1 -> cmult0_4_0/3
  c_to_ri4_0/2 -> delay0_4_0_3/1, delay1_3_0_3/1, delay2_2_0_3/1, delay3_1_0_3/1, delay4_0_0_1/1, delay4_0_0_3/1, delay4_1_0_1/1, delay4_2_0_1/1, delay4_3_0_1/1
  delay0_4_0_3/1 -> cmult0_4_0/4
  cmult0_4_0/1 -> cvrt0_4_0_real/1(din)
  cmult0_4_0/2 -> cvrt0_4_0_imag/1(din)
  cvrt0_4_0_real/1(dout) -> ri_to_c0_4_0/1
  cvrt0_4_0_imag/1(dout) -> ri_to_c0_4_0/2
  ri_to_c0_4_0/1 -> pack0_4/1(in1)
  pack0_4/1(bus_out) -> din0_x_din4*/1
  delay0_5_0_0/1 -> cmult0_5_0/1
  delay0_5_0_1/1 -> cmult0_5_0/2
  c_to_ri5_0/1 -> delay0_5_0_2/1, delay1_4_0_2/1, delay2_3_0_2/1, delay3_2_0_2/1, delay4_1_0_2/1, delay5_0_0_0/1, delay5_0_0_2/1, delay5_1_0_0/1, delay5_2_0_0/1
  delay0_5_0_2/1 -> cmult0_5_0/3
  c_to_ri5_0/2 -> delay0_5_0_3/1, delay1_4_0_3/1, delay2_3_0_3/1, delay3_2_0_3/1, delay4_1_0_3/1, delay5_0_0_1/1, delay5_0_0_3/1, delay5_1_0_1/1, delay5_2_0_1/1
  delay0_5_0_3/1 -> cmult0_5_0/4
  cmult0_5_0/1 -> cvrt0_5_0_real/1(din)
  cmult0_5_0/2 -> cvrt0_5_0_imag/1(din)
  cvrt0_5_0_real/1(dout) -> ri_to_c0_5_0/1
  cvrt0_5_0_imag/1(dout) -> ri_to_c0_5_0/2
  ri_to_c0_5_0/1 -> pack0_5/1(in1)
  pack0_5/1(bus_out) -> din0_x_din5*/1
  delay0_6_0_0/1 -> cmult0_6_0/1
  delay0_6_0_1/1 -> cmult0_6_0/2
  c_to_ri6_0/1 -> delay0_6_0_2/1, delay1_5_0_2/1, delay2_4_0_2/1, delay3_3_0_2/1, delay4_2_0_2/1, delay5_1_0_2/1, delay6_0_0_0/1, delay6_0_0_2/1, delay6_1_0_0/1
  delay0_6_0_2/1 -> cmult0_6_0/3
  c_to_ri6_0/2 -> delay0_6_0_3/1, delay1_5_0_3/1, delay2_4_0_3/1, delay3_3_0_3/1, delay4_2_0_3/1, delay5_1_0_3/1, delay6_0_0_1/1, delay6_0_0_3/1, delay6_1_0_1/1
  delay0_6_0_3/1 -> cmult0_6_0/4
  cmult0_6_0/1 -> cvrt0_6_0_real/1(din)
  cmult0_6_0/2 -> cvrt0_6_0_imag/1(din)
  cvrt0_6_0_real/1(dout) -> ri_to_c0_6_0/1
  cvrt0_6_0_imag/1(dout) -> ri_to_c0_6_0/2
  ri_to_c0_6_0/1 -> pack0_6/1(in1)
  pack0_6/1(bus_out) -> din0_x_din6*/1
  delay0_7_0_0/1 -> cmult0_7_0/1
  delay0_7_0_1/1 -> cmult0_7_0/2
  c_to_ri7_0/1 -> delay0_7_0_2/1, delay1_6_0_2/1, delay2_5_0_2/1, delay3_4_0_2/1, delay4_3_0_2/1, delay5_2_0_2/1, delay6_1_0_2/1, delay7_0_0_0/1, delay7_0_0_2/1
  delay0_7_0_2/1 -> cmult0_7_0/3
  c_to_ri7_0/2 -> delay0_7_0_3/1, delay1_6_0_3/1, delay2_5_0_3/1, delay3_4_0_3/1, delay4_3_0_3/1, delay5_2_0_3/1, delay6_1_0_3/1, delay7_0_0_1/1, delay7_0_0_3/1
  delay0_7_0_3/1 -> cmult0_7_0/4
  cmult0_7_0/1 -> cvrt0_7_0_real/1(din)
  cmult0_7_0/2 -> cvrt0_7_0_imag/1(din)
  cvrt0_7_0_real/1(dout) -> ri_to_c0_7_0/1
  cvrt0_7_0_imag/1(dout) -> ri_to_c0_7_0/2
  ri_to_c0_7_0/1 -> pack0_7/1(in1)
  pack0_7/1(bus_out) -> din0_x_din7*/1
  delay1_0_0_0/1 -> cmult1_0_0/1
  delay1_0_0_1/1 -> cmult1_0_0/2
  delay1_0_0_2/1 -> cmult1_0_0/3
  delay1_0_0_3/1 -> cmult1_0_0/4
  cmult1_0_0/1 -> cvrt1_0_0_real/1(din)
  cmult1_0_0/2 -> cvrt1_0_0_imag/1(din)
  cvrt1_0_0_real/1(dout) -> ri_to_c1_0_0/1
  cvrt1_0_0_imag/1(dout) -> ri_to_c1_0_0/2
  ri_to_c1_0_0/1 -> pack1_0/1(in1)
  pack1_0/1(bus_out) -> din1_x_din1*/1
  delay1_1_0_0/1 -> cmult1_1_0/1
  delay1_1_0_1/1 -> cmult1_1_0/2
  delay1_1_0_2/1 -> cmult1_1_0/3
  delay1_1_0_3/1 -> cmult1_1_0/4
  cmult1_1_0/1 -> cvrt1_1_0_real/1(din)
  cmult1_1_0/2 -> cvrt1_1_0_imag/1(din)
  cvrt1_1_0_real/1(dout) -> ri_to_c1_1_0/1
  cvrt1_1_0_imag/1(dout) -> ri_to_c1_1_0/2
  ri_to_c1_1_0/1 -> pack1_1/1(in1)
  pack1_1/1(bus_out) -> din1_x_din2*/1
  delay1_2_0_0/1 -> cmult1_2_0/1
  delay1_2_0_1/1 -> cmult1_2_0/2
  delay1_2_0_2/1 -> cmult1_2_0/3
  delay1_2_0_3/1 -> cmult1_2_0/4
  cmult1_2_0/1 -> cvrt1_2_0_real/1(din)
  cmult1_2_0/2 -> cvrt1_2_0_imag/1(din)
  cvrt1_2_0_real/1(dout) -> ri_to_c1_2_0/1
  cvrt1_2_0_imag/1(dout) -> ri_to_c1_2_0/2
  ri_to_c1_2_0/1 -> pack1_2/1(in1)
  pack1_2/1(bus_out) -> din1_x_din3*/1
  delay1_3_0_0/1 -> cmult1_3_0/1
  delay1_3_0_1/1 -> cmult1_3_0/2
  delay1_3_0_2/1 -> cmult1_3_0/3
  delay1_3_0_3/1 -> cmult1_3_0/4
  cmult1_3_0/1 -> cvrt1_3_0_real/1(din)
  cmult1_3_0/2 -> cvrt1_3_0_imag/1(din)
  cvrt1_3_0_real/1(dout) -> ri_to_c1_3_0/1
  cvrt1_3_0_imag/1(dout) -> ri_to_c1_3_0/2
  ri_to_c1_3_0/1 -> pack1_3/1(in1)
  pack1_3/1(bus_out) -> din1_x_din4*/1
  delay1_4_0_0/1 -> cmult1_4_0/1
  delay1_4_0_1/1 -> cmult1_4_0/2
  delay1_4_0_2/1 -> cmult1_4_0/3
  delay1_4_0_3/1 -> cmult1_4_0/4
  cmult1_4_0/1 -> cvrt1_4_0_real/1(din)
  cmult1_4_0/2 -> cvrt1_4_0_imag/1(din)
  cvrt1_4_0_real/1(dout) -> ri_to_c1_4_0/1
  cvrt1_4_0_imag/1(dout) -> ri_to_c1_4_0/2
  ri_to_c1_4_0/1 -> pack1_4/1(in1)
  pack1_4/1(bus_out) -> din1_x_din5*/1
  delay1_5_0_0/1 -> cmult1_5_0/1
  delay1_5_0_1/1 -> cmult1_5_0/2
  delay1_5_0_2/1 -> cmult1_5_0/3
  delay1_5_0_3/1 -> cmult1_5_0/4
  cmult1_5_0/1 -> cvrt1_5_0_real/1(din)
  cmult1_5_0/2 -> cvrt1_5_0_imag/1(din)
  cvrt1_5_0_real/1(dout) -> ri_to_c1_5_0/1
  cvrt1_5_0_imag/1(dout) -> ri_to_c1_5_0/2
  ri_to_c1_5_0/1 -> pack1_5/1(in1)
  pack1_5/1(bus_out) -> din1_x_din6*/1
  delay1_6_0_0/1 -> cmult1_6_0/1
  delay1_6_0_1/1 -> cmult1_6_0/2
  delay1_6_0_2/1 -> cmult1_6_0/3
  delay1_6_0_3/1 -> cmult1_6_0/4
  cmult1_6_0/1 -> cvrt1_6_0_real/1(din)
  cmult1_6_0/2 -> cvrt1_6_0_imag/1(din)
  cvrt1_6_0_real/1(dout) -> ri_to_c1_6_0/1
  cvrt1_6_0_imag/1(dout) -> ri_to_c1_6_0/2
  ri_to_c1_6_0/1 -> pack1_6/1(in1)
  pack1_6/1(bus_out) -> din1_x_din7*/1
  delay2_0_0_0/1 -> cmult2_0_0/1
  delay2_0_0_1/1 -> cmult2_0_0/2
  delay2_0_0_2/1 -> cmult2_0_0/3
  delay2_0_0_3/1 -> cmult2_0_0/4
  cmult2_0_0/1 -> cvrt2_0_0_real/1(din)
  cmult2_0_0/2 -> cvrt2_0_0_imag/1(din)
  cvrt2_0_0_real/1(dout) -> ri_to_c2_0_0/1
  cvrt2_0_0_imag/1(dout) -> ri_to_c2_0_0/2
  ri_to_c2_0_0/1 -> pack2_0/1(in1)
  pack2_0/1(bus_out) -> din2_x_din2*/1
  delay2_1_0_0/1 -> cmult2_1_0/1
  delay2_1_0_1/1 -> cmult2_1_0/2
  delay2_1_0_2/1 -> cmult2_1_0/3
  delay2_1_0_3/1 -> cmult2_1_0/4
  cmult2_1_0/1 -> cvrt2_1_0_real/1(din)
  cmult2_1_0/2 -> cvrt2_1_0_imag/1(din)
  cvrt2_1_0_real/1(dout) -> ri_to_c2_1_0/1
  cvrt2_1_0_imag/1(dout) -> ri_to_c2_1_0/2
  ri_to_c2_1_0/1 -> pack2_1/1(in1)
  pack2_1/1(bus_out) -> din2_x_din3*/1
  delay2_2_0_0/1 -> cmult2_2_0/1
  delay2_2_0_1/1 -> cmult2_2_0/2
  delay2_2_0_2/1 -> cmult2_2_0/3
  delay2_2_0_3/1 -> cmult2_2_0/4
  cmult2_2_0/1 -> cvrt2_2_0_real/1(din)
  cmult2_2_0/2 -> cvrt2_2_0_imag/1(din)
  cvrt2_2_0_real/1(dout) -> ri_to_c2_2_0/1
  cvrt2_2_0_imag/1(dout) -> ri_to_c2_2_0/2
  ri_to_c2_2_0/1 -> pack2_2/1(in1)
  pack2_2/1(bus_out) -> din2_x_din4*/1
  delay2_3_0_0/1 -> cmult2_3_0/1
  delay2_3_0_1/1 -> cmult2_3_0/2
  delay2_3_0_2/1 -> cmult2_3_0/3
  delay2_3_0_3/1 -> cmult2_3_0/4
  cmult2_3_0/1 -> cvrt2_3_0_real/1(din)
  cmult2_3_0/2 -> cvrt2_3_0_imag/1(din)
  cvrt2_3_0_real/1(dout) -> ri_to_c2_3_0/1
  cvrt2_3_0_imag/1(dout) -> ri_to_c2_3_0/2
  ri_to_c2_3_0/1 -> pack2_3/1(in1)
  pack2_3/1(bus_out) -> din2_x_din5*/1
  delay2_4_0_0/1 -> cmult2_4_0/1
  delay2_4_0_1/1 -> cmult2_4_0/2
  delay2_4_0_2/1 -> cmult2_4_0/3
  delay2_4_0_3/1 -> cmult2_4_0/4
  cmult2_4_0/1 -> cvrt2_4_0_real/1(din)
  cmult2_4_0/2 -> cvrt2_4_0_imag/1(din)
  cvrt2_4_0_real/1(dout) -> ri_to_c2_4_0/1
  cvrt2_4_0_imag/1(dout) -> ri_to_c2_4_0/2
  ri_to_c2_4_0/1 -> pack2_4/1(in1)
  pack2_4/1(bus_out) -> din2_x_din6*/1
  delay2_5_0_0/1 -> cmult2_5_0/1
  delay2_5_0_1/1 -> cmult2_5_0/2
  delay2_5_0_2/1 -> cmult2_5_0/3
  delay2_5_0_3/1 -> cmult2_5_0/4
  cmult2_5_0/1 -> cvrt2_5_0_real/1(din)
  cmult2_5_0/2 -> cvrt2_5_0_imag/1(din)
  cvrt2_5_0_real/1(dout) -> ri_to_c2_5_0/1
  cvrt2_5_0_imag/1(dout) -> ri_to_c2_5_0/2
  ri_to_c2_5_0/1 -> pack2_5/1(in1)
  pack2_5/1(bus_out) -> din2_x_din7*/1
  delay3_0_0_0/1 -> cmult3_0_0/1
  delay3_0_0_1/1 -> cmult3_0_0/2
  delay3_0_0_2/1 -> cmult3_0_0/3
  delay3_0_0_3/1 -> cmult3_0_0/4
  cmult3_0_0/1 -> cvrt3_0_0_real/1(din)
  cmult3_0_0/2 -> cvrt3_0_0_imag/1(din)
  cvrt3_0_0_real/1(dout) -> ri_to_c3_0_0/1
  cvrt3_0_0_imag/1(dout) -> ri_to_c3_0_0/2
  ri_to_c3_0_0/1 -> pack3_0/1(in1)
  pack3_0/1(bus_out) -> din3_x_din3*/1
  delay3_1_0_0/1 -> cmult3_1_0/1
  delay3_1_0_1/1 -> cmult3_1_0/2
  delay3_1_0_2/1 -> cmult3_1_0/3
  delay3_1_0_3/1 -> cmult3_1_0/4
  cmult3_1_0/1 -> cvrt3_1_0_real/1(din)
  cmult3_1_0/2 -> cvrt3_1_0_imag/1(din)
  cvrt3_1_0_real/1(dout) -> ri_to_c3_1_0/1
  cvrt3_1_0_imag/1(dout) -> ri_to_c3_1_0/2
  ri_to_c3_1_0/1 -> pack3_1/1(in1)
  pack3_1/1(bus_out) -> din3_x_din4*/1
  delay3_2_0_0/1 -> cmult3_2_0/1
  delay3_2_0_1/1 -> cmult3_2_0/2
  delay3_2_0_2/1 -> cmult3_2_0/3
  delay3_2_0_3/1 -> cmult3_2_0/4
  cmult3_2_0/1 -> cvrt3_2_0_real/1(din)
  cmult3_2_0/2 -> cvrt3_2_0_imag/1(din)
  cvrt3_2_0_real/1(dout) -> ri_to_c3_2_0/1
  cvrt3_2_0_imag/1(dout) -> ri_to_c3_2_0/2
  ri_to_c3_2_0/1 -> pack3_2/1(in1)
  pack3_2/1(bus_out) -> din3_x_din5*/1
  delay3_3_0_0/1 -> cmult3_3_0/1
  delay3_3_0_1/1 -> cmult3_3_0/2
  delay3_3_0_2/1 -> cmult3_3_0/3
  delay3_3_0_3/1 -> cmult3_3_0/4
  cmult3_3_0/1 -> cvrt3_3_0_real/1(din)
  cmult3_3_0/2 -> cvrt3_3_0_imag/1(din)
  cvrt3_3_0_real/1(dout) -> ri_to_c3_3_0/1
  cvrt3_3_0_imag/1(dout) -> ri_to_c3_3_0/2
  ri_to_c3_3_0/1 -> pack3_3/1(in1)
  pack3_3/1(bus_out) -> din3_x_din6*/1
  delay3_4_0_0/1 -> cmult3_4_0/1
  delay3_4_0_1/1 -> cmult3_4_0/2
  delay3_4_0_2/1 -> cmult3_4_0/3
  delay3_4_0_3/1 -> cmult3_4_0/4
  cmult3_4_0/1 -> cvrt3_4_0_real/1(din)
  cmult3_4_0/2 -> cvrt3_4_0_imag/1(din)
  cvrt3_4_0_real/1(dout) -> ri_to_c3_4_0/1
  cvrt3_4_0_imag/1(dout) -> ri_to_c3_4_0/2
  ri_to_c3_4_0/1 -> pack3_4/1(in1)
  pack3_4/1(bus_out) -> din3_x_din7*/1
  delay4_0_0_0/1 -> cmult4_0_0/1
  delay4_0_0_1/1 -> cmult4_0_0/2
  delay4_0_0_2/1 -> cmult4_0_0/3
  delay4_0_0_3/1 -> cmult4_0_0/4
  cmult4_0_0/1 -> cvrt4_0_0_real/1(din)
  cmult4_0_0/2 -> cvrt4_0_0_imag/1(din)
  cvrt4_0_0_real/1(dout) -> ri_to_c4_0_0/1
  cvrt4_0_0_imag/1(dout) -> ri_to_c4_0_0/2
  ri_to_c4_0_0/1 -> pack4_0/1(in1)
  pack4_0/1(bus_out) -> din4_x_din4*/1
  delay4_1_0_0/1 -> cmult4_1_0/1
  delay4_1_0_1/1 -> cmult4_1_0/2
  delay4_1_0_2/1 -> cmult4_1_0/3
  delay4_1_0_3/1 -> cmult4_1_0/4
  cmult4_1_0/1 -> cvrt4_1_0_real/1(din)
  cmult4_1_0/2 -> cvrt4_1_0_imag/1(din)
  cvrt4_1_0_real/1(dout) -> ri_to_c4_1_0/1
  cvrt4_1_0_imag/1(dout) -> ri_to_c4_1_0/2
  ri_to_c4_1_0/1 -> pack4_1/1(in1)
  pack4_1/1(bus_out) -> din4_x_din5*/1
  delay4_2_0_0/1 -> cmult4_2_0/1
  delay4_2_0_1/1 -> cmult4_2_0/2
  delay4_2_0_2/1 -> cmult4_2_0/3
  delay4_2_0_3/1 -> cmult4_2_0/4
  cmult4_2_0/1 -> cvrt4_2_0_real/1(din)
  cmult4_2_0/2 -> cvrt4_2_0_imag/1(din)
  cvrt4_2_0_real/1(dout) -> ri_to_c4_2_0/1
  cvrt4_2_0_imag/1(dout) -> ri_to_c4_2_0/2
  ri_to_c4_2_0/1 -> pack4_2/1(in1)
  pack4_2/1(bus_out) -> din4_x_din6*/1
  delay4_3_0_0/1 -> cmult4_3_0/1
  delay4_3_0_1/1 -> cmult4_3_0/2
  delay4_3_0_2/1 -> cmult4_3_0/3
  delay4_3_0_3/1 -> cmult4_3_0/4
  cmult4_3_0/1 -> cvrt4_3_0_real/1(din)
  cmult4_3_0/2 -> cvrt4_3_0_imag/1(din)
  cvrt4_3_0_real/1(dout) -> ri_to_c4_3_0/1
  cvrt4_3_0_imag/1(dout) -> ri_to_c4_3_0/2
  ri_to_c4_3_0/1 -> pack4_3/1(in1)
  pack4_3/1(bus_out) -> din4_x_din7*/1
  delay5_0_0_0/1 -> cmult5_0_0/1
  delay5_0_0_1/1 -> cmult5_0_0/2
  delay5_0_0_2/1 -> cmult5_0_0/3
  delay5_0_0_3/1 -> cmult5_0_0/4
  cmult5_0_0/1 -> cvrt5_0_0_real/1(din)
  cmult5_0_0/2 -> cvrt5_0_0_imag/1(din)
  cvrt5_0_0_real/1(dout) -> ri_to_c5_0_0/1
  cvrt5_0_0_imag/1(dout) -> ri_to_c5_0_0/2
  ri_to_c5_0_0/1 -> pack5_0/1(in1)
  pack5_0/1(bus_out) -> din5_x_din5*/1
  delay5_1_0_0/1 -> cmult5_1_0/1
  delay5_1_0_1/1 -> cmult5_1_0/2
  delay5_1_0_2/1 -> cmult5_1_0/3
  delay5_1_0_3/1 -> cmult5_1_0/4
  cmult5_1_0/1 -> cvrt5_1_0_real/1(din)
  cmult5_1_0/2 -> cvrt5_1_0_imag/1(din)
  cvrt5_1_0_real/1(dout) -> ri_to_c5_1_0/1
  cvrt5_1_0_imag/1(dout) -> ri_to_c5_1_0/2
  ri_to_c5_1_0/1 -> pack5_1/1(in1)
  pack5_1/1(bus_out) -> din5_x_din6*/1
  delay5_2_0_0/1 -> cmult5_2_0/1
  delay5_2_0_1/1 -> cmult5_2_0/2
  delay5_2_0_2/1 -> cmult5_2_0/3
  delay5_2_0_3/1 -> cmult5_2_0/4
  cmult5_2_0/1 -> cvrt5_2_0_real/1(din)
  cmult5_2_0/2 -> cvrt5_2_0_imag/1(din)
  cvrt5_2_0_real/1(dout) -> ri_to_c5_2_0/1
  cvrt5_2_0_imag/1(dout) -> ri_to_c5_2_0/2
  ri_to_c5_2_0/1 -> pack5_2/1(in1)
  pack5_2/1(bus_out) -> din5_x_din7*/1
  delay6_0_0_0/1 -> cmult6_0_0/1
  delay6_0_0_1/1 -> cmult6_0_0/2
  delay6_0_0_2/1 -> cmult6_0_0/3
  delay6_0_0_3/1 -> cmult6_0_0/4
  cmult6_0_0/1 -> cvrt6_0_0_real/1(din)
  cmult6_0_0/2 -> cvrt6_0_0_imag/1(din)
  cvrt6_0_0_real/1(dout) -> ri_to_c6_0_0/1
  cvrt6_0_0_imag/1(dout) -> ri_to_c6_0_0/2
  ri_to_c6_0_0/1 -> pack6_0/1(in1)
  pack6_0/1(bus_out) -> din6_x_din6*/1
  delay6_1_0_0/1 -> cmult6_1_0/1
  delay6_1_0_1/1 -> cmult6_1_0/2
  delay6_1_0_2/1 -> cmult6_1_0/3
  delay6_1_0_3/1 -> cmult6_1_0/4
  cmult6_1_0/1 -> cvrt6_1_0_real/1(din)
  cmult6_1_0/2 -> cvrt6_1_0_imag/1(din)
  cvrt6_1_0_real/1(dout) -> ri_to_c6_1_0/1
  cvrt6_1_0_imag/1(dout) -> ri_to_c6_1_0/2
  ri_to_c6_1_0/1 -> pack6_1/1(in1)
  pack6_1/1(bus_out) -> din6_x_din7*/1
  delay7_0_0_0/1 -> cmult7_0_0/1
  delay7_0_0_1/1 -> cmult7_0_0/2
  delay7_0_0_2/1 -> cmult7_0_0/3
  delay7_0_0_3/1 -> cmult7_0_0/4
  cmult7_0_0/1 -> cvrt7_0_0_real/1(din)
  cmult7_0_0/2 -> cvrt7_0_0_imag/1(din)
  cvrt7_0_0_real/1(dout) -> ri_to_c7_0_0/1
  cvrt7_0_0_imag/1(dout) -> ri_to_c7_0_0/2
  ri_to_c7_0_0/1 -> pack7_0/1(in1)
  pack7_0/1(bus_out) -> din7_x_din7*/1
